simulink model "TCC_MODEL"  (R2025a)
settings: Solver=ode23t  StartTime=0.0  StopTime=1010  FixedStep=0.01  RelTol=1e-3
values from neighbouring files (symbols this model uses):
  HYST = 2    [parametros_componentes.m]
  I_table = [  1.6305773075253425 ... (first row only)    [parametros_componentes.m]
  Icc = -0.000008    (= -8e-06)    [parametros_componentes.m]
  IDD = 25e-6    (= 2.5e-05)    [parametros_componentes.m]
  Ildo = -0.00007    (= -7e-05)    [parametros_componentes.m]
  Iload = 0    [parametros_componentes.m]
  Inicio_da_descarga = 1000    [parametros_componentes.m]
  Inicio_do_curto = 10    [parametros_componentes.m]
  R_curto = 0.5    [parametros_componentes.m]
  R_descarga = (V_BATT_TOTAL+12)/corrente_Max_bat    (= 8.05)    [parametros_componentes.m]
  R_inicial = 0.18    [parametros_componentes.m]
  R_trip = 64.8    [parametros_componentes.m]
  SOC_inicial = 1    [parametros_componentes.m]
  t_table = [  93.22913720326267 ... (first row only)    [parametros_componentes.m]
  tempo_simu_curto = 70    [parametros_componentes.m]
  tempo_simu_descarga = 20    [parametros_componentes.m]
  tempo_simu_temp = 50000    [parametros_componentes.m]
  TSET = 55    [parametros_componentes.m]
  VDD = 3.3    [parametros_componentes.m]
libraries: fl_lib x29, nesl_utility x21, batt_lib x12, ee_lib x2, simulink x1, BatteryEstimators x1
(part 1 of 2)
settings Model: Creator=marce  LastModifiedBy=marce

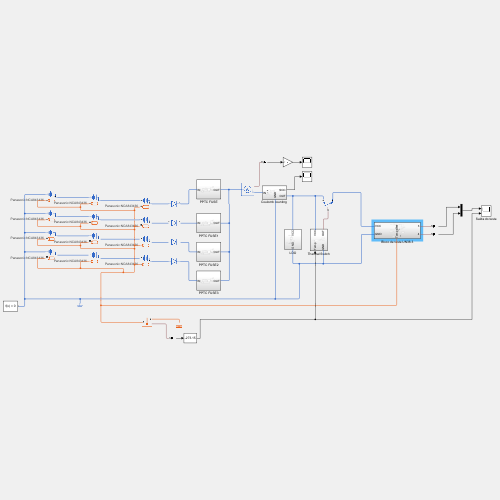
[thumbnail: Simulink's stored preview of the top-level diagram]
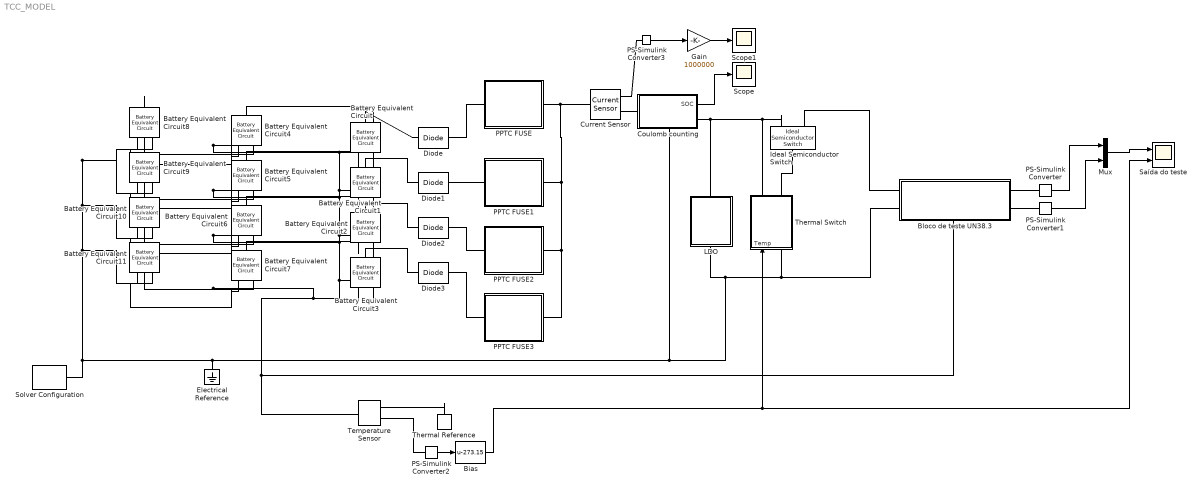
== system TCC_MODEL ==
  Battery Equivalent Circuit : batt_lib/Cells/Battery Equivalent Circuit  PartSpecification="{\"CollectionId\":\"SimscapeBattery\",\"CollectionVersion\":\"1.0.0\",\"DatasetId\":\"Panasonic|NCA843436|simscape.battery.batteryEquivalentCircuit\",\"DisplayName\":\"Panasonic:NCA843436\"}"  BatteryCapacity=1.354 % Datasheet derived hr*A  ThermalModel=simscape.battery.enum.cells.BatteryThermalModel.LumpedThermalMass  ExtrapolationMethod=simscape.enum.extrapolation.linear  SOCBreakpoints=[0 0.01 0.02 0.03 0.04 0.05 0.06 0.07 0.08 0.09 0.1 0.11 0.12 0.13 0.14 0.15 0.16 0.17 0.18 0.19 0.2 0.21 0.22 0.23 0.24 0.25 0.26 0.27 0.28 0.29 0.3 0.31 0.32 0.33 0.34 0.35 0.36 0.37 0.38 0.39 0.4 0.41 0.42 0.43 0.44 0.45 0.46 0.47 0.48 0.49 0.5 0.51 0.52 0.53 0.54 0.55 0.56 0.57 0.58 0.59 0.6 0.61 0.62 0.63 0.64 0.65 0.66 0.67 0.68 0.69 0.7 0.71 0.72 0.73 0.74 0.75 0.76 0.77 0.78 0.79 0.8 0.81 0.82 0.83 0.84 0.85 0.86 0.87 0.88 0.89 0.9 0.91 0.92 0.93 0.94 0.95 0.96 0.97 0.98 0.99 1] % Datasheet derived  TemperatureBreakpoints=[-10 0 10 25 45 60] % Datasheet derived degC  OpenCircuitVoltage=[2.817 2.94537 3.0182 3.08984 3.15197 3.18868 3.22389 3.25188 3.27953 3.3028 3.32214 3.34136 3.36247 3.37682 3.38851 3.4018 3.4147 3.42636 3.43803 3.44822 3.45549 3.46277 3.47005 3.47732 3.4846 3.49328 3.49997 3.50631 3.51243 3.51855 3.52468 3.5308 3.53692 3.54304 3.54917 3.55568 3.56257 3.56948 3.57636 3.58289 3.58942 3.59595 3.60248 3.60901 3.61554 3.62207 3.62861 3.63511 3.64233 3.65 3.65825 3.6665 3.67476 3.68301 3.69126 3.69952 3.70777 3.71583 3.72334 3.73246 3.74258 3.75276 3.76295 3.77313 3.78331 3.7935 3.80368 3.81459 3.82556 3.83654 3.84646 3.85584 3.86522 3.87454 3.8835 3.89255 3.9016 3.91065 3.91971 3.92884 3.93875 3.95021 3.96167 3.97312 3.98443 3.99549 4.00655 4.01783 4.0295 4.04093 4.05161 4.06166 4.07171 4.08185 4.09229 4.10286 4.11335 4.12383 4.13431 4.1515 4.17492] % Datasheet derived V  OpenCircuitVoltageThermal=[2.817 2.817 2.817 2.817 2.817 2.817;2.94537 2.94537 2.94537 2.94537 2.94537 2.94537;3.0182 3.0182 3.0182 3.0182 3.0182 3.0182;3.08984 3.08984 3.08984 3.08984 3.08984 3.08984;3.15197 3.15197 3.15197 3.15197 3.15197 3.15197;3.18868 3.18868 3.18868 3.18868 3.18868 3.18868;3.22389 3.22389 3.22389 3.22389 3.22389 3.22389;3.25188 3.25188 3.25188 3.25188 3.25188 3.25188;3.27953 3.27953 3.27953 3.27953 3.27953 3.27953;3.3028 3.3028 3.3028 3.3028 3.3028 3.3028;3.32214 3.32214 3.32214 3.32214 3.32214 3.32214;3.34136 3.34136 3.34136 3.34136 3.34136 3.34136;3.36247 3.36247 3.36247 3.36247 3.36247 3.36247;3.37682 3.37682 3.37682 3.37682 3.37682 3.37682;3.38851 3.38851 3.38851 3.38851 3.38851 3.38851;3.4018 3.4018 3.4018 3.4018 3.4018 3.4018;3.4147 3.4147 3.4147 3.4147 3.4147 3.4147;3.42636 3.42636 3.42636 3.42636 3.42636 3.42636;3.43803 3.43803 3.43803 3.43803 3.43803 3.43803;3.44822 3.44822 3.44822 3.44822 3.44822 3.44822;3.45549 3.45549 3.45549 3.45549 3.45549 3.45549;3.46277 3.46277 3.46277 3.46277 3.46277 3.46277;3.47005 3.47005 3.47005 3.47005 3.47005 3.47005;3.47732 3.47732 3.47732 3.47732 3.47732 3.47732;3.4846 3.4846 3.4846 3.4846 3.4846 3.4846;3.49328 3.49328 3.49328 3.49328 3.49328 3.49328;3.49997 3.49997 3.49997 3.49997 3.49997 3.49997;3.50631 3.50631 3.50631 3.50631 3.50631 3.50631;3.51243 3.51243 3.51243 3.51243 3.51243 3.51243;3.51855 3.51855 3.51855 3.51855 3.51855 3.51855;3.52468 3.52468 3.52468 3.52468 3.52468 3.52468;3.5308 3.5308 3.5308 3.5308 3.5308 3.5308;3.53692 3.53692 3.53692 3.53692 3.53692 3.53692;3.54304 3.54304 3.54304 3.54304 3.54304 3.54304;3.54917 3.54917 3.54917 3.54917 3.54917 3.54917;3.55568 3.55568 3.55568 3.55568 3.55568 3.55568;3.56257 3.56257 3.56257 3.56257 3.56257 3.56257;3.56948 3.56948 3.56948 3.56948 3.56948 3.56948;3.57636 3.57636 3.57636 3.57636 3.57636 3.57636;3.58289 3.58289 3.58289 3.58289 3.58289 3.58289;3.58942 3.58942 3.58942 3.58942 3.58942 3.58942;3.59595 3.59595 3.59595 3.59595 3.59595 3.59595;3.60248 3.60248 3.60248 3.60248 3.60248 3.60248;3.60901 3.60901 3.60901 3.60901 3.60901 3.60901;3.61554 3.61554 3.61554 3.61554 3.61554 3.61554;3.62207 3.62207 3.62207 3.62207 3.62207 3.62207;3.62861 3.62861 3.62861 3.62861 3.62861 3.62861;3.63511 3.63511 3.63511 3.63511 3.63511 3.63511;3.64233 3.64233 3.64233 3.64233 3.64233 3.64233;3.65 3.65 3.65 3.65 3.65 3.65;3.65825 3.65825 3.65825 3.65825 3.65825 3.65825;3.6665 3.6665 3.6665 3.6665 3.6665 3.6665;3.67476 3.67476 3.67476 3.67476 3.67476 3.67476;3.68301 3.68301 3.68301 3.68301 3.68301 3.68301;3.69126 3.69126 3.69126 3.69126 3.69126 3.69126;3.69952 3.69952 3.69952 3.69952 3.69952 3.69952;3.70777 3.70777 3.70777 3.70777 3.70777 3.70777;3.71583 3.71583 3.71583 3.71583 3.71583 3.71583;3.72334 3.72334 3.72334 3.72334 3.72334 3.72334;3.73246 3.73246 3.73246 3.73246 3.73246 3.73246;3.74258 3.74258 3.74258 3.74258 3.74258 3.74258;3.75276 3.75276 3.75276 3.75276 3.75276 3.75276;3.76295 3.76295 3.76295 3.76295 3.76295 3.76295;3.77313 3.77313 3.77313 3.77313 3.77313 3.77313;3.78331 3.78331 3.78331 3.78331 3.78331 3.78331;3.7935 3.7935 3.7935 3.7935 3.7935 3.7935;3.80368 3.80368 3.80368 3.80368 3.80368 3.80368;3.81459 3.81459 3.81459 3.81459 3.81459 3.81459;3.82556 3.82556 3.82556 3.82556 3.82556 3.82556;3.83654 3.83654 3.83654 3.83654 3.83654 3.83654;3.84646 3.84646 3.84646 3.84646 3.84646 3.84646;3.85584 3.85584 3.85584 3.85584 3.85584 3.85584;3.86522 3.86522 3.86522 3.86522 3.86522 3.86522;3.87454 3.87454 3.87454 3.87454 3.87454 3.87454;3.8835 3.8835 3.8835 3.8835 3.8835 3.8835;3.89255 3.89255 3.89255 3.89255 3.89255 3.89255;3.9016 3.9016 3.9016 3.9016 3.9016 3.9016;3.91065 3.91065 3.91065 3.91065 3.91065 3.91065;3.91971 3.91971 3.91971 3.91971 3.91971 3.91971;3.92884 3.92884 3.92884 3.92884 3.92884 3.92884;3.93875 3.93875 3.93875 3.93875 3.93875 3.93875;3.95021 3.95021 3.95021 3.95021 3.95021 3.95021;3.96167 3.96167 3.96167 3.96167 3.96167 3.96167;3.97312 3.97312 3.97312 3.97312 3.97312 3.97312;3.98443 3.98443 3.98443 3.98443 3.98443 3.98443;3.99549 ...(+748 chars)] % Datasheet derived V  VoltageRange=[2.25 Inf] % Datasheet derived V  HysteresisModel=simscape.battery.enum.cells.HysteresisModel.none  MaximumHysteresisVoltage=[0, 0, 0, 0, 0, 0, 0] % Parameter not set V  InstantaneousHysteresisVoltage=[0, 0, 0, 0, 0, 0, 0] % Parameter not set V  HysteresisRate=0.1 % Parameter not set  MaximumHysteresisVoltageThermal=[0, 0, 0; 0, 0, 0; 0, 0, 0; 0, 0, 0; 0, 0, 0; 0, 0, 0; 0, 0, 0] % Parameter not set V  InstantaneousHysteresisVoltageThermal=[0, 0, 0; 0, 0, 0; 0, 0, 0; 0, 0, 0; 0, 0, 0; 0, 0, 0; 0, 0, 0] % Parameter not set V  HysteresisRateThermal=0.1 % Parameter not set  ResistanceSOCBreakpoints=[0 0.01 0.02 0.03 0.04 0.05 0.06 0.07 0.08 0.09 0.1 0.11 0.12 0.13 0.14 0.15 0.16 0.17 0.18 0.19 0.2 0.21 0.22 0.23 0.24 0.25 0.26 0.27 0.28 0.29 0.3 0.31 0.32 0.33 0.34 0.35 0.36 0.37 0.38 0.39 0.4 0.41 0.42 0.43 0.44 0.45 0.46 0.47 0.48 0.49 0.5 0.51 0.52 0.53 0.54 0.55 0.56 0.57 0.58 0.59 0.6 0.61 0.62 0.63 0.64 0.65 0.66 0.67 0.68 0.69 0.7 0.71 0.72 0.73 0.74 0.75 0.76 0.77 0.78 0.79 0.8 0.81 0.82 0.83 0.84 0.85 0.86 0.87 0.88 0.89 0.9 0.91 0.92 0.93 0.94 0.95 0.96 0.97 0.98 0.99 1] % Datasheet derived  ResistanceTemperatureBreakpoints=[-10 0 10 25 45 60] % Datasheet derived degC  ResistanceCurrentBreakpoints=[-1, 0, 1] % Parameter not set A  CurrentDependence=simscape.battery.enum.cells.CurrentDependence.Disabled  R0=[0.31638 0.3243 0.30647 0.2881 0.26534 0.23483 0.21466 0.1963 0.19065 0.18321 0.17517 0.17035 0.1686 0.16602 0.16263 0.16182 0.16098 0.16003 0.15908 0.15746 0.15485 0.15224 0.14963 0.14702 0.14441 0.14408 0.14309 0.14204 0.14098 0.13992 0.13886 0.13779 0.13673 0.13567 0.13461 0.13373 0.13328 0.13287 0.13246 0.13202 0.13158 0.13114 0.1307 0.13026 0.12982 0.12938 0.12894 0.12846 0.12829 0.12823 0.12821 0.1282 0.12818 0.12817 0.12815 0.12814 0.12812 0.12779 0.12659 0.12613 0.1261 0.12607 0.12605 0.12602 0.126 0.12598 0.12595 0.12709 0.12835 0.1296 0.13037 0.13088 0.1314 0.13182 0.13158 0.13136 0.13113 0.1309 0.13069 0.13059 0.13086 0.13184 0.13283 0.13381 0.13455 0.1349 0.13525 0.13561 0.13601 0.1363 0.13601 0.1347 0.13339 0.13211 0.13099 0.12903 0.12626 0.1235 0.12073 0.11181 0.10295] % Datasheet derived Ohm  R0I=[.0117, .0085, .009; .011, .0085, .009; .0114, .0087, .0092; .0107, .0082, .0088; .0107, .0083, .0091; .0113, .0085, .0089; .0116, .0085, .0089] % Parameter not set Ohm  R0Thermal=[1.5461 1.75516 2.11759 0.31638 0.46651 0.23498;1.5461 1.99954 2.27305 0.3243 0.34615 0.09965;1.5461 1.92281 2.1374 0.30647 0.20343 0.05211;1.5461 1.84609 2.00176 0.2881 0.15069 0.02648;1.5461 1.76937 1.86611 0.26534 0.12351 0.03545;1.5461 1.69264 1.73046 0.23483 0.10579 0.0319;1.5461 1.61592 1.59482 0.21466 0.09923 0.03983;1.5461 1.5392 1.45917 0.1963 0.0958 0.05105;1.5461 1.46247 1.32352 0.19065 0.10282 0.06344;1.5461 1.38575 1.18787 0.18321 0.10641 0.07241;1.5461 1.30902 1.05223 0.17517 0.10811 0.07828;1.5461 1.2323 0.91658 0.17035 0.11082 0.08499;1.5461 1.15558 0.78093 0.1686 0.11501 0.09321;1.50339 1.07885 0.64529 0.16602 0.11389 0.09611;1.46067 1.00213 0.52896 0.16263 0.11281 0.09693;1.41796 0.92541 0.45732 0.16182 0.1148 0.09886;1.37525 0.84868 0.40356 0.16098 0.11649 0.10041;1.33254 0.77196 0.35633 0.16003 0.1172 0.10099;1.28982 0.69523 0.32513 0.15908 0.11792 0.10158;1.24711 0.61749 0.29756 0.15746 0.11748 0.101;1.2044 0.5576 0.27681 0.15485 0.11475 0.09814;1.16169 0.50708 0.25953 0.15224 0.11202 0.09528;1.11897 0.46758 0.24304 0.14963 0.11054 0.09242;1.07626 0.43256 0.23145 0.14702 0.10939 0.09016;1.03355 0.40213 0.21986 0.14441 0.10825 0.08946;0.99084 0.37836 0.21479 0.14408 0.10821 0.08986;0.94812 0.35585 0.21092 0.14309 0.1066 0.08869;0.90541 0.33652 0.20677 0.14204 0.10481 0.08725;0.8627 0.32218 0.20275 0.14098 0.10391 0.08564;0.81999 0.30785 0.19912 0.13992 0.10301 0.08404;0.77727 0.29756 0.19549 0.13886 0.1021 0.08274;0.73457 0.28818 0.19186 0.13779 0.10125 0.08295;0.69186 0.2788 0.1889 0.13673 0.10088 0.08317;0.65043 0.27154 0.18649 0.13567 0.10051 0.08339;0.60913 0.26481 0.18408 0.13461 0.10013 0.0836;0.57538 0.25838 0.18198 0.13373 0.10007 0.08413;0.5481 0.25225 0.18022 0.13328 0.10029 0.08494;0.52084 0.24869 0.17996 0.13287 0.10054 0.08577;0.49467 0.24569 0.17968 0.13246 0.10076 0.08658;0.47265 0.24242 0.17912 0.13202 0.10071 0.08711;0.45063 0.23914 0.17856 0.13158 0.10065 0.08708;0.43278 0.23587 0.17801 0.13114 0.10056 0.08706;0.42113 0.23372 0.17745 0.1307 0.09993 0.08703;0.40948 0.23194 0.17689 0.13026 0.09931 0.087;0.39802 0.23016 0.17625 0.12982 0.09869 0.08698;0.3895 0.22838 0.17554 0.12938 0.09807 0.08695;0.38098 0.2266 0.17484 0.12894 0.09745 0.08692;0.37243 0.2248 0.17411 0.12846 0.09681 0.08688;0.36446 0.22399 0.17395 0.12829 0.09673 0.08739;0.35683 0.2238 0.17413 0.12823 0.097 0.08826;0.35467 0.22407 0.17478 0.12821 0.09771 0.08958;0.35251 0.22433 0.17543 0.1282 0.098 0.09079;0.35035 0.2246 0.17607 0.12818 0.09829 0.09028;0.34819 0.22487 0.17654 0.12817 0.09857 0.08977;0.34604 0.22513 0.17577 0.12815 0.09886 0.08925;0.34388 0.2254 0.175 0.12814 0.09915 0.08874;0.34172 0.22541 0.17423 0.12812 0.09944 0.08823;0.3394 0.22519 0.17331 0.12779 0.09957 0.08756;0.33667 0.22454 0.17196 0.12659 0.09928 0.08647;0.33518 0.22514 0.17187 0.12613 0.10014 0.08664;0.33524 0.22653 0.17256 0.1261 0.10082 0.08759;0.33556 0.22797 0.1733 0.12607 0.10155 0.0885;0.33589 0.22941 0.17405 0.12605 0.10227 0.08918;0.33622 0.23086 0.17484 0.12602 0.103 0.08985;0.33655 0.2323 0.1758 0.126 0.10373 0.09053;0.33688 0.23374 0.17676 0.12598 0.10446 0.0912;0.33721 0.23499 0.17772 0.12595 0.10519 0.09188;0.3381 0.23639 0.17924 0.12709 0.10648 0.09312;0.33905 0.23784 0.18082 0.12835 0.10783 0.09441;0.34 0.23929 0.18241 0.1296 0.10918 0.09571;0.34031 0.23991 0.18316 0.13037 0.1097 0.09618;0.34036 0.24011 0.18349 0.13088 0.1098 0.09608;0.3404 0.24031 0.18382 0.1314 0.10989 0.09597;0.3404 0.24047 0.1841 0.13182 0.10986 0.09581;0.34011 0.24033 0.1841 0.13158 0.10953 0.09535;0.33989 0.24027 0.18422 0.13136 0.10929 0.09498;0.34006 0.24021 0.18463 0.13113 0.10904 0.09461;0.34112 0.24015 0.18505 0.1309 0.1088 0.09423;0.34219 0.24057 0.18547 0.13069 0.10855 0.09385;0.34331 0.24158 0.18594 0.13059 0.10837 0.09322;0.34505 0.2432 0.18703 0.13086 0.10748 0.0932;0.348 0.24604 0.18933 0.13184 0.10774 0.09438;0.35095 0.24887 0.19163 0.13283 0.108 0.09557;0.35389 0.25171 0.19393 0.13381 0.10826 0.09676;0.35814 0.25442 0.19611 0.13455 0.1084 0.09783 ...(+755 chars)] % Datasheet derived Ohm  R0ThermalI=repmat([.0117, .0085, .009; .011, .0085, .009; .0114, .0087, .0092; .0107, .0082, .0088; .0107, .0083, .0091; .0113, .0085, .0089; .0116, .0085, .0089], 1, 1, 3) % Parameter not set Ohm  DischargeR0=[.0085, .0085, .0087, .0082, .0083, .0085, .0085] % Parameter not set Ohm  ChargeR0=[.0085, .0085, .0087, .0082, .0083, .0085, .0085] % Parameter not set Ohm  ChargeR0Thermal=[.0117, .0085, .009; .011, .0085, .009; .0114, .0087, .0092; .0107, .0082, .0088; .0107, .0083, .0091; .0113, .0085, .0089; .0116, .0085, .0089] % Parameter not set Ohm  DischargeR0Thermal=[.0117, .0085, .009; .011, .0085, .009; .0114, .0087, .0092; .0107, .0082, .0088; .0107, .0083, .0091; .0113, .0085, .0089; .0116, .0085, .0089] % Parameter not set Ohm  RCPairs=simscape.battery.enum.cells.RCPairs.noDynamics  R1=[.0029, .0024, .0026, .0016, .0023, .0018, .0017] % Parameter not set Ohm  Tau1=[36, 45, 105, 29, 77, 33, 39] % Parameter not set s  R2=[.0029, .0024, .0026, .0016, .0023, .0018, .0017] % Parameter not set Ohm  Tau2=[36, 45, 105, 29, 77, 33, 39] % Parameter not set s  R3=[.0029, .0024, .0026, .0016, .0023, .0018, .0017] % Parameter not set Ohm  Tau3=[36, 45, 105, 29, 77, 33, 39] % Parameter not set s  R1I=[.0109, .0029, .0013; .0069, .0024, .0012; .0047, .0026, .0013; .0034, .0016, .001; .0033, .0023, .0014; .0033, .0018, .0011; .0028, .0017, .0011] % Parameter not set Ohm  Tau1I=[20, 36, 39; 31, 45, 39; 109, 105, 61; 36, 29, 26; 59, 77, 67; 40, 33, 29; 25, 39, 33] % Parameter not set s  R2I=[.0109, .0029, .0013; .0069, .0024, .0012; .0047, .0026, .0013; .0034, .0016, .001; .0033, .0023, .0014; .0033, .0018, .0011; .0028, .0017, .0011] % Parameter not set Ohm  Tau2I=[20, 36, 39; 31, 45, 39; 109, 105, 61; 36, 29, 26; 59, 77, 67; 40, 33, 29; 25, 39, 33] % Parameter not set s  R3I=[.0109, .0029, .0013; .0069, .0024, .0012; .0047, .0026, .0013; .0034, .0016, .001; .0033, .0023, .0014; .0033, .0018, .0011; .0028, .0017, .0011] % Parameter not set Ohm  Tau3I=[20, 36, 39; 31, 45, 39; 109, 105, 61; 36, 29, 26; 59, 77, 67; 40, 33, 29; 25, 39, 33] % Parameter not set s  DischargeR1=[.0029, .0024, .0026, .0016, .0023, .0018, .0017] % Parameter not set Ohm  DischargeTau1=[36, 45, 105, 29, 77, 33, 39] % Parameter not set s  ChargeR1=[.0029, .0024, .0026, .0016, .0023, .0018, .0017] % Parameter not set Ohm  ChargeTau1=[36, 45, 105, 29, 77, 33, 39] % Parameter not set s  DischargeR2=[.0029, .0024, .0026, .0016, .0023, .0018, .0017] % Parameter not set Ohm  DischargeTau2=[36, 45, 105, 29, 77, 33, 39] % Parameter not set s  ChargeR2=[.0029, .0024, .0026, .0016, .0023, .0018, .0017] % Parameter not set Ohm  ChargeTau2=[36, 45, 105, 29, 77, 33, 39] % Parameter not set s  DischargeR3=[.0029, .0024, .0026, .0016, .0023, .0018, .0017] % Parameter not set Ohm  DischargeTau3=[36, 45, 105, 29, 77, 33, 39] % Parameter not set s  ChargeR3=[.0029, .0024, .0026, .0016, .0023, .0018, .0017] % Parameter not set Ohm  ChargeTau3=[36, 45, 105, 29, 77, 33, 39] % Parameter not set s  R1Thermal=[.0109, .0029, .0013; .0069, .0024, .0012; .0047, .0026, .0013; .0034, .0016, .001; .0033, .0023, .0014; .0033, .0018, .0011; .0028, .0017, .0011] % Parameter not set Ohm  Tau1Thermal=[20, 36, 39; 31, 45, 39; 109, 105, 61; 36, 29, 26; 59, 77, 67; 40, 33, 29; 25, 39, 33] % Parameter not set s  R2Thermal=[.0109, .0029, .0013; .0069, .0024, .0012; .0047, .0026, .0013; .0034, .0016, .001; .0033, .0023, .0014; .0033, .0018, .0011; .0028, .0017, .0011] % Parameter not set Ohm  Tau2Thermal=[20, 36, 39; 31, 45, 39; 109, 105, 61; 36, 29, 26; 59, 77, 67; 40, 33, 29; 25, 39, 33] % Parameter not set s  R3Thermal=[.0109, .0029, .0013; .0069, .0024, .0012; .0047, .0026, .0013; .0034, .0016, .001; .0033, .0023, .0014; .0033, .0018, .0011; .0028, .0017, .0011] % Parameter not set Ohm  Tau3Thermal=[20, 36, 39; 31, 45, 39; 109, 105, 61; 36, 29, 26; 59, 77, 67; 40, 33, 29; 25, 39, 33] % Parameter not set s  R1ThermalI=repmat([.0109, .0029, .0013; .0069, .0024, .0012; .0047, .0026, .0013; .0034, .0016, .001; .0033, .0023, .0014; .0033, .0018, .0011; .0028, .0017, .0011], 1, 1, 3) % Parameter not set Ohm  Tau1ThermalI=repmat([20, 36, 39; 31, 45, 39; 109, 105, 61; 36, 29, 26; 59, 77, 67; 40, 33, 29; 25, 39, 33], 1, 1, 3) % Parameter not set s  R2ThermalI=repmat([.0109, .0029, .0013; .0069, .0024, .0012; .0047, .0026, .0013; .0034, .0016, .001; .0033, .0023, .0014; .0033, .0018, .0011; .0028, .0017, .0011], 1, 1, 3) % Parameter not set Ohm  Tau2ThermalI=repmat([20, 36, 39; 31, 45, 39; 109, 105, 61; 36, 29, 26; 59, 77, 67; 40, 33, 29; 25, 39, 33], 1, 1, 3) % Parameter not set s  R3ThermalI=repmat([.0109, .0029, .0013; .0069, .0024, .0012; .0047, .0026, .0013; .0034, .0016, .001; .0033, .0023, .0014; .0033, .0018, .0011; .0028, .0017, .0011], 1, 1, 3) % Parameter not set Ohm  Tau3ThermalI=repmat([20, 36, 39; 31, 45, 39; 109, 105, 61; 36, 29, 26; 59, 77, 67; 40, 33, 29; 25, 39, 33], 1, 1, 3) % Parameter not set s  DischargeR1Thermal=[.0109, .0029, .0013; .0069, .0024, .0012; .0047, .0026, .0013; .0034, .0016, .001; .0033, .0023, .0014; .0033, .0018, .0011; .0028, .0017, .0011] % Parameter not set Ohm  DischargeTau1Thermal=[20, 36, 39; 31, 45, 39; 109, 105, 61; 36, 29, 26; 59, 77, 67; 40, 33, 29; 25, 39, 33] % Parameter not set s  ChargeR1Thermal=[.0109, .0029, .0013; .0069, .0024, .0012; .0047, .0026, .0013; .0034, .0016, .001; .0033, .0023, .0014; .0033, .0018, .0011; .0028, .0017, .0011] % Parameter not set Ohm  ChargeTau1Thermal=[20, 36, 39; 31, 45, 39; 109, 105, 61; 36, 29, 26; 59, 77, 67; 40, 33, 29; 25, 39, 33] % Parameter not set s  DischargeR2Thermal=[.0109, .0029, .0013; .0069, .0024, .0012; .0047, .0026, .0013; .0034, .0016, .001; .0033, .0023, .0014; .0033, .0018, .0011; .0028, .0017, .0011] % Parameter not set Ohm  DischargeTau2Thermal=[20, 36, 39; 31, 45, 39; 109, 105, 61; 36, 29, 26; 59, 77, 67; 40, 33, 29; 25, 39, 33] % Parameter not set s  ChargeR2Thermal=[.0109, .0029, .0013; .0069, .0024, .0012; .0047, .0026, .0013; .0034, .0016, .001; .0033, .0023, .0014; .0033, .0018, .0011; .0028, .0017, .0011] % Parameter not set Ohm  ChargeTau2Thermal=[20, 36, 39; 31, 45, 39; 109, 105, 61; 36, 29, 26; 59, 77, 67; 40, 33, 29; 25, 39, 33] % Parameter not set s  DischargeR3Thermal=[.0109, .0029, .0013; .0069, .0024, .0012; .0047, .0026, .0013; .0034, .0016, .001; .0033, .0023, .0014; .0033, .0018, .0011; .0028, .0017, .0011] % Parameter not set Ohm  DischargeTau3Thermal=[20, 36, 39; 31, 45, 39; 109, 105, 61; 36, 29, 26; 59, 77, 67; 40, 33, 29; 25, 39, 33] % Parameter not set s  ChargeR3Thermal=[.0109, .0029, .0013; .0069, .0024, .0012; .0047, .0026, .0013; .0034, .0016, .001; .0033, .0023, .0014; .0033, .0018, .0011; .0028, .0017, .0011] % Parameter not set Ohm  ChargeTau3Thermal=[20, 36, 39; 31, 45, 39; 109, 105, 61; 36, 29, 26; 59, 77, 67; 40, 33, 29; 25, 39, 33] % Parameter not set s  SelfDischargeResistor=simscape.battery.enum.cells.BatteryEnable.Disabled  SelfDischargeR=7e3 % Parameter not set Ohm  SelfDischargeRThermal=[8000, 7000, 6000] % Parameter not set Ohm  CyclingAgingMethod=simscape.battery.enum.cells.CyclingAgingMethod.tableN  CycleCalculationMethod=simscape.battery.enum.cells.CycleCalculationMethod.EquivalentCycles  NumDisCycles=100 % Parameter not set  OCVChange=0 % Parameter not set  R0Change=0 % Parameter not set  CapacityChange=0 % Parameter not set  SelfDischargeRChange=0 % Parameter not set  R1Change=0 % Parameter not set  R2Change=0 % Parameter not set  R3Change=0 % Parameter not set  NumDisCyclesBreakpoints=[0 7 13 19 25 31 37 43 49 55 61 67 73 79 85 91 97 103 109 115 121 127 133 139 145 151 157 163 169 175 181 187 193 199 205 211 217 223 229 235 241 247 253 259 265 271 277 283 289 295 301 307 313 319 325 331 337 343 349 355 361 367 373 379 385 391 397 403 409 415 421 427 433 439 445 451 457 463 469 475 481 487 493 499] % Datasheet derived  AgingTemperatureBreakpoints=[298.15, 323.15] % Parameter not set K  AgingCurrentBreakpoints=[-.1, -.5, -5] % Parameter not set A  OCVChangeVec=[0 -0.2056 -0.4112 -0.602 -0.7529 -0.9041 -1.0234 -1.116 -1.2087 -1.3013 -1.3939 -1.4865 -1.5404 -1.5936 -1.6468 -1.7 -1.7534 -1.807 -1.8607 -1.9143 -1.972 -2.0316 -2.0912 -2.1507 -2.2103 -2.2687 -2.3264 -2.3842 -2.442 -2.4996 -2.5474 -2.5914 -2.6354 -2.6795 -2.7235 -2.7676 -2.8116 -2.8556 -2.8997 -2.9437 -2.9899 -3.057 -3.1273 -3.1975 -3.2718 -3.347 -3.4222 -3.4977 -3.5744 -3.6428 -3.6945 -3.7461 -3.7966 -3.8466 -3.8965 -3.9465 -3.9964 -4.0461 -4.0951 -4.1498 -4.2072 -4.2646 -4.322 -4.3794 -4.4368 -4.4942 -4.5515 -4.61 -4.6685 -4.7269 -4.7854 -4.844 -4.9032 -4.9624 -5.0216 -5.0808 -5.1413 -5.2041 -5.2668 -5.3295 -5.3922 -5.455 -5.5177 -5.5804] % Datasheet derived  OCVChangeThermal=[0, 0; 0, 0; 0, 0; 0, 0] % Parameter not set  R0ChangeVec=[0 0 0 0 0 0 0 0 0 0 0 0 0 0 0 0 0 0 0 0 0 0 0 0 0 0 0 0 0 0 0 0 0 0 0 0 0 0 0 0 0 0 0 0 0 0 0 0 0 0 0 0 0 0 0 0 0 0 0 0 0 0 0 0 0 0 0 0 0 0 0 0 0 0 0 0 0 0 0 0 0 0 0 0] % Parameter assumed  R0ChangeThermal=[0, 0; 0, 0; 0, 0; 0, 0] % Parameter not set  R0ChangeThermalI=repmat(0, 4, 2, 3) % Parameter not set  R0CyclingChangeInitialTarget=0 % Parameter not set  CapacityChangeVec=[0 -0.367 -0.733 -1.1 -1.466 -1.834 -2.202 -2.571 -2.94 -3.309 -3.678 -4.047 -4.261 -4.473 -4.685 -4.897 -5.109 -5.32 -5.532 -5.744 -5.972 -6.21 -6.448 -6.686 -6.924 -7.162 -7.4 -7.638 -7.876 -8.114 -8.313 -8.496 -8.679 -8.862 -9.045 -9.228 -9.411 -9.593 -9.776 -9.959 -10.142 -10.405 -10.679 -10.954 -11.228 -11.503 -11.777 -12.052 -12.326 -12.571 -12.756 -12.941 -13.126 -13.311 -13.496 -13.681 -13.866 -14.051 -14.235 -14.442 -14.659 -14.875 -15.092 -15.308 -15.525 -15.741 -15.958 -16.175 -16.391 -16.607 -16.822 -17.038 -17.254 -17.47 -17.685 -17.901 -18.122 -18.35 -18.579 -18.807 -19.036 -19.265 -19.493 -19.722] % Datasheet derived  CapacityChangeThermal=[0, 0; 0, 0; 0, 0; 0, 0] % Parameter not set  CapacityChangeThermalI=repmat(0, 4, 2, 3) % Parameter not set  CapacityCyclingChangeInitialTarget=0 % Parameter not set  SelfDischargeRChangeVec=[0, 0, 0, 0] % Parameter not set  SelfDischargeRChangeThermal=[0, 0; 0, 0; 0, 0; 0, 0] % Parameter not set  SelfDischargeRChangeThermalI=repmat(0, 4, 2, 3) % Parameter not set  SelfDischargeRCyclingChangeInitialTarget=0 % Parameter not set  R1ChangeVec=[0, 0, 0, 0] % Parameter not set  R1ChangeThermal=[0, 0; 0, 0; 0, 0; 0, 0] % Parameter not set  R1ChangeThermalI=repmat(0, 4, 2, 3) % Parameter not set  R1CyclingChangeInitialTarget=0 % Parameter not set  R2ChangeVec=[0, 0, 0, 0] % Parameter not set  R2ChangeThermal=[0, 0; 0, 0; 0, 0; 0, 0] % Parameter not set  R2ChangeThermalI=repmat(0, 4, 2, 3) % Parameter not set  R2CyclingChangeInitialTarget=0 % Parameter not set  R3ChangeVec=[0, 0, 0, 0] % Parameter not set  R3ChangeThermal=[0, 0; 0, 0; 0, 0; 0, 0] % Parameter not set  R3ChangeThermalI=repmat(0, 4, 2, 3) % Parameter not set  R3CyclingChangeInitialTarget=0 % Parameter not set  CalendarAgeResistance=simscape.battery.enum.cells.BatteryEnable.Disabled  CalendarAgeCapacity=simscape.battery.enum.cells.BatteryEnable.Disabled  CalendarAgingMethod=simscape.battery.enum.cells.CalendarAgingMethod.equation  StorageVariable=simscape.battery.enum.cells.StorageVariable.OCV  OCVDuringStorage=0.9 % Parameter not set  SOCDuringStorage=0.6 % Parameter not set  StorageTimeIntervals=[0] % Parameter not set d  StorageTemperatures=[273] % Parameter not set K  ResistanceScalingOCV=2.2134e6 % Parameter not set  ResistanceScalingOCVOffset=1.632e6 % Parameter not set  ResistanceExponentialIncrease=0.515833569 % Parameter not set V  ResistanceTimeExponent=0.75 % Parameter not set  ResistanceAgeTemperatureBreakpoints=[273.15, 298.15, 323.15] % Parameter not set K  ResistanceAgeTimeBreakpoints=[0, 90, 180, 270] % Parameter not set d  PercentResistanceChange=[0, 0, 0] % Parameter not set  ResistanceTimeBreakpoints=100 % Parameter not set d  PercentResistanceChangeThermal=[0, 0, 0; 0, 0, 0; 0, 0, 0; 0, 0, 0] % Parameter not set  CapacityScalingOCV=1.5097e07 % Parameter not set  CapacityScalingOCVOffset=8.3625e06 % Parameter not set  CapacityExponentialIncrease=0.6011 % Parameter not set V  CapacityTimeExponent=0.75 % Parameter not set  CapacityAgeTemperatureBreakpoints=[273.15, 298.15, 323.15] % Parameter not set K  CapacityAgeTimeBreakpoints=[0, 90, 180, 270] % Parameter not set d  PercentCapacityChange=[0, 0, 0] % Parameter not set  CapacityTimeBreakpoints=100 % Parameter not set d  PercentCapacityChangeThermal=[0, 0, 0; 0, 0, 0; 0, 0, 0; 0, 0, 0] % Parameter not set  SimulationTemperature=298.15 % Parameter not set K  BatteryThermalMass=20.7 % Parameter assumed J/K  NumThermalModels=6 % Parameter not set  ThermalConductivityZ=18 % Parameter not set W/(K*m)  CrossSectionalAreaXY=0.000286 m^2  Height=0.036 m  ReversibleHeatModel=simscape.battery.enum.cells.ReversibleHeatModel.Disabled  EntropicCoefficient=[0, 0, 0, 0, 0, 0, 0] % Parameter not set mV/K  CurrentDirectionality=simscape.battery.enum.cells.BatteryEnable.Disabled  stateOfCharge_specify=off  stateOfCharge_priority=High  stateOfCharge=1  stateOfCharge_nominal_specify=off  stateOfCharge_nominal_value=1  stateOfCharge_nominal_unit=1  batteryVoltage_specify=off  batteryVoltage_priority=Low  batteryVoltage=3 V  batteryVoltage_nominal_specify=off  batteryVoltage_nominal_value=1  batteryVoltage_nominal_unit=V  batteryCurrent_specify=off  batteryCurrent_priority=None  batteryCurrent=0 A  batteryCurrent_nominal_specify=off  batteryCurrent_nominal_value=1  batteryCurrent_nominal_unit=A  numCycles_specify=off  numCycles_priority=High  numCycles=0  numCycles_nominal_specify=off  numCycles_nominal_value=1  numCycles_nominal_unit=1  batteryTemperature_specify=off  batteryTemperature_priority=High  batteryTemperature=298.15 K  batteryTemperature_nominal_specify=off  batteryTemperature_nominal_value=1  batteryTemperature_nominal_unit=K  hysteresisState_specify=off  hysteresisState_priority=High  hysteresisState=0  hysteresisState_nominal_specify=off  hysteresisState_nominal_value=1  hysteresisState_nominal_unit=1  isExothermFaulted_specify=off  isExothermFaulted_priority=None  isExothermFaulted=0  isExothermFaulted_nominal_specify=off  isExothermFaulted_nominal_value=1  isExothermFaulted_nominal_unit=1  reactionHeatRate_specify=off  reactionHeatRate_priority=None  reactionHeatRate=0 W  reactionHeatRate_nominal_specify=off  reactionHeatRate_nominal_value=1  reactionHeatRate_nominal_unit=W  reactionExtent_specify=off  reactionExtent_priority=None  reactionExtent=0  reactionExtent_nominal_specify=off  reactionExtent_nominal_value=1  reactionExtent_nominal_unit=1
      settings: AttributesFormatString=Panasonic:NCA843436  InternalSimscapePortConfiguration="{\"Bottom\":[{\"id\":\"n\",\"label\":\"-\",\"type\":\"foundation.electrical.electrical\"},{\"id\":\"H\",\"label\":\"H\",\"type\":\"foundation.thermal.thermal\"}],\"Left\":[],\"Right\":[],\"Top\":[{\"id\":\"p\",\"label\":\"+\",\"type\":\"foundation.electrical.electrical\"}]}"
  Battery Equivalent Circuit{1..3,5..7,9..11} (9 alike) : batt_lib/Cells/Battery Equivalent Circuit  PartSpecification="{\"CollectionId\":\"SimscapeBattery\",\"CollectionVersion\":\"1.0.0\",\"DatasetId\":\"Panasonic|NCA843436|simscape.battery.batteryEquivalentCircuit\",\"DisplayName\":\"Panasonic:NCA843436\"}"  BatteryCapacity=1.354 % Datasheet derived hr*A  ThermalModel=simscape.battery.enum.cells.BatteryThermalModel.LumpedThermalMass  ExtrapolationMethod=simscape.enum.extrapolation.linear  SOCBreakpoints=[0 0.01 0.02 0.03 0.04 0.05 0.06 0.07 0.08 0.09 0.1 0.11 0.12 0.13 0.14 0.15 0.16 0.17 0.18 0.19 0.2 0.21 0.22 0.23 0.24 0.25 0.26 0.27 0.28 0.29 0.3 0.31 0.32 0.33 0.34 0.35 0.36 0.37 0.38 0.39 0.4 0.41 0.42 0.43 0.44 0.45 0.46 0.47 0.48 0.49 0.5 0.51 0.52 0.53 0.54 0.55 0.56 0.57 0.58 0.59 0.6 0.61 0.62 0.63 0.64 0.65 0.66 0.67 0.68 0.69 0.7 0.71 0.72 0.73 0.74 0.75 0.76 0.77 0.78 0.79 0.8 0.81 0.82 0.83 0.84 0.85 0.86 0.87 0.88 0.89 0.9 0.91 0.92 0.93 0.94 0.95 0.96 0.97 0.98 0.99 1] % Datasheet derived  TemperatureBreakpoints=[-10 0 10 25 45 60] % Datasheet derived degC  OpenCircuitVoltage=[2.817 2.94537 3.0182 3.08984 3.15197 3.18868 3.22389 3.25188 3.27953 3.3028 3.32214 3.34136 3.36247 3.37682 3.38851 3.4018 3.4147 3.42636 3.43803 3.44822 3.45549 3.46277 3.47005 3.47732 3.4846 3.49328 3.49997 3.50631 3.51243 3.51855 3.52468 3.5308 3.53692 3.54304 3.54917 3.55568 3.56257 3.56948 3.57636 3.58289 3.58942 3.59595 3.60248 3.60901 3.61554 3.62207 3.62861 3.63511 3.64233 3.65 3.65825 3.6665 3.67476 3.68301 3.69126 3.69952 3.70777 3.71583 3.72334 3.73246 3.74258 3.75276 3.76295 3.77313 3.78331 3.7935 3.80368 3.81459 3.82556 3.83654 3.84646 3.85584 3.86522 3.87454 3.8835 3.89255 3.9016 3.91065 3.91971 3.92884 3.93875 3.95021 3.96167 3.97312 3.98443 3.99549 4.00655 4.01783 4.0295 4.04093 4.05161 4.06166 4.07171 4.08185 4.09229 4.10286 4.11335 4.12383 4.13431 4.1515 4.17492] % Datasheet derived V  OpenCircuitVoltageThermal=[2.817 2.817 2.817 2.817 2.817 2.817;2.94537 2.94537 2.94537 2.94537 2.94537 2.94537;3.0182 3.0182 3.0182 3.0182 3.0182 3.0182;3.08984 3.08984 3.08984 3.08984 3.08984 3.08984;3.15197 3.15197 3.15197 3.15197 3.15197 3.15197;3.18868 3.18868 3.18868 3.18868 3.18868 3.18868;3.22389 3.22389 3.22389 3.22389 3.22389 3.22389;3.25188 3.25188 3.25188 3.25188 3.25188 3.25188;3.27953 3.27953 3.27953 3.27953 3.27953 3.27953;3.3028 3.3028 3.3028 3.3028 3.3028 3.3028;3.32214 3.32214 3.32214 3.32214 3.32214 3.32214;3.34136 3.34136 3.34136 3.34136 3.34136 3.34136;3.36247 3.36247 3.36247 3.36247 3.36247 3.36247;3.37682 3.37682 3.37682 3.37682 3.37682 3.37682;3.38851 3.38851 3.38851 3.38851 3.38851 3.38851;3.4018 3.4018 3.4018 3.4018 3.4018 3.4018;3.4147 3.4147 3.4147 3.4147 3.4147 3.4147;3.42636 3.42636 3.42636 3.42636 3.42636 3.42636;3.43803 3.43803 3.43803 3.43803 3.43803 3.43803;3.44822 3.44822 3.44822 3.44822 3.44822 3.44822;3.45549 3.45549 3.45549 3.45549 3.45549 3.45549;3.46277 3.46277 3.46277 3.46277 3.46277 3.46277;3.47005 3.47005 3.47005 3.47005 3.47005 3.47005;3.47732 3.47732 3.47732 3.47732 3.47732 3.47732;3.4846 3.4846 3.4846 3.4846 3.4846 3.4846;3.49328 3.49328 3.49328 3.49328 3.49328 3.49328;3.49997 3.49997 3.49997 3.49997 3.49997 3.49997;3.50631 3.50631 3.50631 3.50631 3.50631 3.50631;3.51243 3.51243 3.51243 3.51243 3.51243 3.51243;3.51855 3.51855 3.51855 3.51855 3.51855 3.51855;3.52468 3.52468 3.52468 3.52468 3.52468 3.52468;3.5308 3.5308 3.5308 3.5308 3.5308 3.5308;3.53692 3.53692 3.53692 3.53692 3.53692 3.53692;3.54304 3.54304 3.54304 3.54304 3.54304 3.54304;3.54917 3.54917 3.54917 3.54917 3.54917 3.54917;3.55568 3.55568 3.55568 3.55568 3.55568 3.55568;3.56257 3.56257 3.56257 3.56257 3.56257 3.56257;3.56948 3.56948 3.56948 3.56948 3.56948 3.56948;3.57636 3.57636 3.57636 3.57636 3.57636 3.57636;3.58289 3.58289 3.58289 3.58289 3.58289 3.58289;3.58942 3.58942 3.58942 3.58942 3.58942 3.58942;3.59595 3.59595 3.59595 3.59595 3.59595 3.59595;3.60248 3.60248 3.60248 3.60248 3.60248 3.60248;3.60901 3.60901 3.60901 3.60901 3.60901 3.60901;3.61554 3.61554 3.61554 3.61554 3.61554 3.61554;3.62207 3.62207 3.62207 3.62207 3.62207 3.62207;3.62861 3.62861 3.62861 3.62861 3.62861 3.62861;3.63511 3.63511 3.63511 3.63511 3.63511 3.63511;3.64233 3.64233 3.64233 3.64233 3.64233 3.64233;3.65 3.65 3.65 3.65 3.65 3.65;3.65825 3.65825 3.65825 3.65825 3.65825 3.65825;3.6665 3.6665 3.6665 3.6665 3.6665 3.6665;3.67476 3.67476 3.67476 3.67476 3.67476 3.67476;3.68301 3.68301 3.68301 3.68301 3.68301 3.68301;3.69126 3.69126 3.69126 3.69126 3.69126 3.69126;3.69952 3.69952 3.69952 3.69952 3.69952 3.69952;3.70777 3.70777 3.70777 3.70777 3.70777 3.70777;3.71583 3.71583 3.71583 3.71583 3.71583 3.71583;3.72334 3.72334 3.72334 3.72334 3.72334 3.72334;3.73246 3.73246 3.73246 3.73246 3.73246 3.73246;3.74258 3.74258 3.74258 3.74258 3.74258 3.74258;3.75276 3.75276 3.75276 3.75276 3.75276 3.75276;3.76295 3.76295 3.76295 3.76295 3.76295 3.76295;3.77313 3.77313 3.77313 3.77313 3.77313 3.77313;3.78331 3.78331 3.78331 3.78331 3.78331 3.78331;3.7935 3.7935 3.7935 3.7935 3.7935 3.7935;3.80368 3.80368 3.80368 3.80368 3.80368 3.80368;3.81459 3.81459 3.81459 3.81459 3.81459 3.81459;3.82556 3.82556 3.82556 3.82556 3.82556 3.82556;3.83654 3.83654 3.83654 3.83654 3.83654 3.83654;3.84646 3.84646 3.84646 3.84646 3.84646 3.84646;3.85584 3.85584 3.85584 3.85584 3.85584 3.85584;3.86522 3.86522 3.86522 3.86522 3.86522 3.86522;3.87454 3.87454 3.87454 3.87454 3.87454 3.87454;3.8835 3.8835 3.8835 3.8835 3.8835 3.8835;3.89255 3.89255 3.89255 3.89255 3.89255 3.89255;3.9016 3.9016 3.9016 3.9016 3.9016 3.9016;3.91065 3.91065 3.91065 3.91065 3.91065 3.91065;3.91971 3.91971 3.91971 3.91971 3.91971 3.91971;3.92884 3.92884 3.92884 3.92884 3.92884 3.92884;3.93875 3.93875 3.93875 3.93875 3.93875 3.93875;3.95021 3.95021 3.95021 3.95021 3.95021 3.95021;3.96167 3.96167 3.96167 3.96167 3.96167 3.96167;3.97312 3.97312 3.97312 3.97312 3.97312 3.97312;3.98443 3.98443 3.98443 3.98443 3.98443 3.98443;3.99549 ...(+748 chars)] % Datasheet derived V  VoltageRange=[2.25 Inf] % Datasheet derived V  HysteresisModel=simscape.battery.enum.cells.HysteresisModel.none  MaximumHysteresisVoltage=[0, 0, 0, 0, 0, 0, 0] % Parameter not set V  InstantaneousHysteresisVoltage=[0, 0, 0, 0, 0, 0, 0] % Parameter not set V  HysteresisRate=0.1 % Parameter not set  MaximumHysteresisVoltageThermal=[0, 0, 0; 0, 0, 0; 0, 0, 0; 0, 0, 0; 0, 0, 0; 0, 0, 0; 0, 0, 0] % Parameter not set V  InstantaneousHysteresisVoltageThermal=[0, 0, 0; 0, 0, 0; 0, 0, 0; 0, 0, 0; 0, 0, 0; 0, 0, 0; 0, 0, 0] % Parameter not set V  HysteresisRateThermal=0.1 % Parameter not set  ResistanceSOCBreakpoints=[0 0.01 0.02 0.03 0.04 0.05 0.06 0.07 0.08 0.09 0.1 0.11 0.12 0.13 0.14 0.15 0.16 0.17 0.18 0.19 0.2 0.21 0.22 0.23 0.24 0.25 0.26 0.27 0.28 0.29 0.3 0.31 0.32 0.33 0.34 0.35 0.36 0.37 0.38 0.39 0.4 0.41 0.42 0.43 0.44 0.45 0.46 0.47 0.48 0.49 0.5 0.51 0.52 0.53 0.54 0.55 0.56 0.57 0.58 0.59 0.6 0.61 0.62 0.63 0.64 0.65 0.66 0.67 0.68 0.69 0.7 0.71 0.72 0.73 0.74 0.75 0.76 0.77 0.78 0.79 0.8 0.81 0.82 0.83 0.84 0.85 0.86 0.87 0.88 0.89 0.9 0.91 0.92 0.93 0.94 0.95 0.96 0.97 0.98 0.99 1] % Datasheet derived  ResistanceTemperatureBreakpoints=[-10 0 10 25 45 60] % Datasheet derived degC  ResistanceCurrentBreakpoints=[-1, 0, 1] % Parameter not set A  CurrentDependence=simscape.battery.enum.cells.CurrentDependence.Disabled  R0=[0.31638 0.3243 0.30647 0.2881 0.26534 0.23483 0.21466 0.1963 0.19065 0.18321 0.17517 0.17035 0.1686 0.16602 0.16263 0.16182 0.16098 0.16003 0.15908 0.15746 0.15485 0.15224 0.14963 0.14702 0.14441 0.14408 0.14309 0.14204 0.14098 0.13992 0.13886 0.13779 0.13673 0.13567 0.13461 0.13373 0.13328 0.13287 0.13246 0.13202 0.13158 0.13114 0.1307 0.13026 0.12982 0.12938 0.12894 0.12846 0.12829 0.12823 0.12821 0.1282 0.12818 0.12817 0.12815 0.12814 0.12812 0.12779 0.12659 0.12613 0.1261 0.12607 0.12605 0.12602 0.126 0.12598 0.12595 0.12709 0.12835 0.1296 0.13037 0.13088 0.1314 0.13182 0.13158 0.13136 0.13113 0.1309 0.13069 0.13059 0.13086 0.13184 0.13283 0.13381 0.13455 0.1349 0.13525 0.13561 0.13601 0.1363 0.13601 0.1347 0.13339 0.13211 0.13099 0.12903 0.12626 0.1235 0.12073 0.11181 0.10295] % Datasheet derived Ohm  R0I=[.0117, .0085, .009; .011, .0085, .009; .0114, .0087, .0092; .0107, .0082, .0088; .0107, .0083, .0091; .0113, .0085, .0089; .0116, .0085, .0089] % Parameter not set Ohm  R0Thermal=[1.5461 1.75516 2.11759 0.31638 0.46651 0.23498;1.5461 1.99954 2.27305 0.3243 0.34615 0.09965;1.5461 1.92281 2.1374 0.30647 0.20343 0.05211;1.5461 1.84609 2.00176 0.2881 0.15069 0.02648;1.5461 1.76937 1.86611 0.26534 0.12351 0.03545;1.5461 1.69264 1.73046 0.23483 0.10579 0.0319;1.5461 1.61592 1.59482 0.21466 0.09923 0.03983;1.5461 1.5392 1.45917 0.1963 0.0958 0.05105;1.5461 1.46247 1.32352 0.19065 0.10282 0.06344;1.5461 1.38575 1.18787 0.18321 0.10641 0.07241;1.5461 1.30902 1.05223 0.17517 0.10811 0.07828;1.5461 1.2323 0.91658 0.17035 0.11082 0.08499;1.5461 1.15558 0.78093 0.1686 0.11501 0.09321;1.50339 1.07885 0.64529 0.16602 0.11389 0.09611;1.46067 1.00213 0.52896 0.16263 0.11281 0.09693;1.41796 0.92541 0.45732 0.16182 0.1148 0.09886;1.37525 0.84868 0.40356 0.16098 0.11649 0.10041;1.33254 0.77196 0.35633 0.16003 0.1172 0.10099;1.28982 0.69523 0.32513 0.15908 0.11792 0.10158;1.24711 0.61749 0.29756 0.15746 0.11748 0.101;1.2044 0.5576 0.27681 0.15485 0.11475 0.09814;1.16169 0.50708 0.25953 0.15224 0.11202 0.09528;1.11897 0.46758 0.24304 0.14963 0.11054 0.09242;1.07626 0.43256 0.23145 0.14702 0.10939 0.09016;1.03355 0.40213 0.21986 0.14441 0.10825 0.08946;0.99084 0.37836 0.21479 0.14408 0.10821 0.08986;0.94812 0.35585 0.21092 0.14309 0.1066 0.08869;0.90541 0.33652 0.20677 0.14204 0.10481 0.08725;0.8627 0.32218 0.20275 0.14098 0.10391 0.08564;0.81999 0.30785 0.19912 0.13992 0.10301 0.08404;0.77727 0.29756 0.19549 0.13886 0.1021 0.08274;0.73457 0.28818 0.19186 0.13779 0.10125 0.08295;0.69186 0.2788 0.1889 0.13673 0.10088 0.08317;0.65043 0.27154 0.18649 0.13567 0.10051 0.08339;0.60913 0.26481 0.18408 0.13461 0.10013 0.0836;0.57538 0.25838 0.18198 0.13373 0.10007 0.08413;0.5481 0.25225 0.18022 0.13328 0.10029 0.08494;0.52084 0.24869 0.17996 0.13287 0.10054 0.08577;0.49467 0.24569 0.17968 0.13246 0.10076 0.08658;0.47265 0.24242 0.17912 0.13202 0.10071 0.08711;0.45063 0.23914 0.17856 0.13158 0.10065 0.08708;0.43278 0.23587 0.17801 0.13114 0.10056 0.08706;0.42113 0.23372 0.17745 0.1307 0.09993 0.08703;0.40948 0.23194 0.17689 0.13026 0.09931 0.087;0.39802 0.23016 0.17625 0.12982 0.09869 0.08698;0.3895 0.22838 0.17554 0.12938 0.09807 0.08695;0.38098 0.2266 0.17484 0.12894 0.09745 0.08692;0.37243 0.2248 0.17411 0.12846 0.09681 0.08688;0.36446 0.22399 0.17395 0.12829 0.09673 0.08739;0.35683 0.2238 0.17413 0.12823 0.097 0.08826;0.35467 0.22407 0.17478 0.12821 0.09771 0.08958;0.35251 0.22433 0.17543 0.1282 0.098 0.09079;0.35035 0.2246 0.17607 0.12818 0.09829 0.09028;0.34819 0.22487 0.17654 0.12817 0.09857 0.08977;0.34604 0.22513 0.17577 0.12815 0.09886 0.08925;0.34388 0.2254 0.175 0.12814 0.09915 0.08874;0.34172 0.22541 0.17423 0.12812 0.09944 0.08823;0.3394 0.22519 0.17331 0.12779 0.09957 0.08756;0.33667 0.22454 0.17196 0.12659 0.09928 0.08647;0.33518 0.22514 0.17187 0.12613 0.10014 0.08664;0.33524 0.22653 0.17256 0.1261 0.10082 0.08759;0.33556 0.22797 0.1733 0.12607 0.10155 0.0885;0.33589 0.22941 0.17405 0.12605 0.10227 0.08918;0.33622 0.23086 0.17484 0.12602 0.103 0.08985;0.33655 0.2323 0.1758 0.126 0.10373 0.09053;0.33688 0.23374 0.17676 0.12598 0.10446 0.0912;0.33721 0.23499 0.17772 0.12595 0.10519 0.09188;0.3381 0.23639 0.17924 0.12709 0.10648 0.09312;0.33905 0.23784 0.18082 0.12835 0.10783 0.09441;0.34 0.23929 0.18241 0.1296 0.10918 0.09571;0.34031 0.23991 0.18316 0.13037 0.1097 0.09618;0.34036 0.24011 0.18349 0.13088 0.1098 0.09608;0.3404 0.24031 0.18382 0.1314 0.10989 0.09597;0.3404 0.24047 0.1841 0.13182 0.10986 0.09581;0.34011 0.24033 0.1841 0.13158 0.10953 0.09535;0.33989 0.24027 0.18422 0.13136 0.10929 0.09498;0.34006 0.24021 0.18463 0.13113 0.10904 0.09461;0.34112 0.24015 0.18505 0.1309 0.1088 0.09423;0.34219 0.24057 0.18547 0.13069 0.10855 0.09385;0.34331 0.24158 0.18594 0.13059 0.10837 0.09322;0.34505 0.2432 0.18703 0.13086 0.10748 0.0932;0.348 0.24604 0.18933 0.13184 0.10774 0.09438;0.35095 0.24887 0.19163 0.13283 0.108 0.09557;0.35389 0.25171 0.19393 0.13381 0.10826 0.09676;0.35814 0.25442 0.19611 0.13455 0.1084 0.09783 ...(+755 chars)] % Datasheet derived Ohm  R0ThermalI=repmat([.0117, .0085, .009; .011, .0085, .009; .0114, .0087, .0092; .0107, .0082, .0088; .0107, .0083, .0091; .0113, .0085, .0089; .0116, .0085, .0089], 1, 1, 3) % Parameter not set Ohm  DischargeR0=[.0085, .0085, .0087, .0082, .0083, .0085, .0085] % Parameter not set Ohm  ChargeR0=[.0085, .0085, .0087, .0082, .0083, .0085, .0085] % Parameter not set Ohm  ChargeR0Thermal=[.0117, .0085, .009; .011, .0085, .009; .0114, .0087, .0092; .0107, .0082, .0088; .0107, .0083, .0091; .0113, .0085, .0089; .0116, .0085, .0089] % Parameter not set Ohm  DischargeR0Thermal=[.0117, .0085, .009; .011, .0085, .009; .0114, .0087, .0092; .0107, .0082, .0088; .0107, .0083, .0091; .0113, .0085, .0089; .0116, .0085, .0089] % Parameter not set Ohm  RCPairs=simscape.battery.enum.cells.RCPairs.noDynamics  R1=[.0029, .0024, .0026, .0016, .0023, .0018, .0017] % Parameter not set Ohm  Tau1=[36, 45, 105, 29, 77, 33, 39] % Parameter not set s  R2=[.0029, .0024, .0026, .0016, .0023, .0018, .0017] % Parameter not set Ohm  Tau2=[36, 45, 105, 29, 77, 33, 39] % Parameter not set s  R3=[.0029, .0024, .0026, .0016, .0023, .0018, .0017] % Parameter not set Ohm  Tau3=[36, 45, 105, 29, 77, 33, 39] % Parameter not set s  R1I=[.0109, .0029, .0013; .0069, .0024, .0012; .0047, .0026, .0013; .0034, .0016, .001; .0033, .0023, .0014; .0033, .0018, .0011; .0028, .0017, .0011] % Parameter not set Ohm  Tau1I=[20, 36, 39; 31, 45, 39; 109, 105, 61; 36, 29, 26; 59, 77, 67; 40, 33, 29; 25, 39, 33] % Parameter not set s  R2I=[.0109, .0029, .0013; .0069, .0024, .0012; .0047, .0026, .0013; .0034, .0016, .001; .0033, .0023, .0014; .0033, .0018, .0011; .0028, .0017, .0011] % Parameter not set Ohm  Tau2I=[20, 36, 39; 31, 45, 39; 109, 105, 61; 36, 29, 26; 59, 77, 67; 40, 33, 29; 25, 39, 33] % Parameter not set s  R3I=[.0109, .0029, .0013; .0069, .0024, .0012; .0047, .0026, .0013; .0034, .0016, .001; .0033, .0023, .0014; .0033, .0018, .0011; .0028, .0017, .0011] % Parameter not set Ohm  Tau3I=[20, 36, 39; 31, 45, 39; 109, 105, 61; 36, 29, 26; 59, 77, 67; 40, 33, 29; 25, 39, 33] % Parameter not set s  DischargeR1=[.0029, .0024, .0026, .0016, .0023, .0018, .0017] % Parameter not set Ohm  DischargeTau1=[36, 45, 105, 29, 77, 33, 39] % Parameter not set s  ChargeR1=[.0029, .0024, .0026, .0016, .0023, .0018, .0017] % Parameter not set Ohm  ChargeTau1=[36, 45, 105, 29, 77, 33, 39] % Parameter not set s  DischargeR2=[.0029, .0024, .0026, .0016, .0023, .0018, .0017] % Parameter not set Ohm  DischargeTau2=[36, 45, 105, 29, 77, 33, 39] % Parameter not set s  ChargeR2=[.0029, .0024, .0026, .0016, .0023, .0018, .0017] % Parameter not set Ohm  ChargeTau2=[36, 45, 105, 29, 77, 33, 39] % Parameter not set s  DischargeR3=[.0029, .0024, .0026, .0016, .0023, .0018, .0017] % Parameter not set Ohm  DischargeTau3=[36, 45, 105, 29, 77, 33, 39] % Parameter not set s  ChargeR3=[.0029, .0024, .0026, .0016, .0023, .0018, .0017] % Parameter not set Ohm  ChargeTau3=[36, 45, 105, 29, 77, 33, 39] % Parameter not set s  R1Thermal=[.0109, .0029, .0013; .0069, .0024, .0012; .0047, .0026, .0013; .0034, .0016, .001; .0033, .0023, .0014; .0033, .0018, .0011; .0028, .0017, .0011] % Parameter not set Ohm  Tau1Thermal=[20, 36, 39; 31, 45, 39; 109, 105, 61; 36, 29, 26; 59, 77, 67; 40, 33, 29; 25, 39, 33] % Parameter not set s  R2Thermal=[.0109, .0029, .0013; .0069, .0024, .0012; .0047, .0026, .0013; .0034, .0016, .001; .0033, .0023, .0014; .0033, .0018, .0011; .0028, .0017, .0011] % Parameter not set Ohm  Tau2Thermal=[20, 36, 39; 31, 45, 39; 109, 105, 61; 36, 29, 26; 59, 77, 67; 40, 33, 29; 25, 39, 33] % Parameter not set s  R3Thermal=[.0109, .0029, .0013; .0069, .0024, .0012; .0047, .0026, .0013; .0034, .0016, .001; .0033, .0023, .0014; .0033, .0018, .0011; .0028, .0017, .0011] % Parameter not set Ohm  Tau3Thermal=[20, 36, 39; 31, 45, 39; 109, 105, 61; 36, 29, 26; 59, 77, 67; 40, 33, 29; 25, 39, 33] % Parameter not set s  R1ThermalI=repmat([.0109, .0029, .0013; .0069, .0024, .0012; .0047, .0026, .0013; .0034, .0016, .001; .0033, .0023, .0014; .0033, .0018, .0011; .0028, .0017, .0011], 1, 1, 3) % Parameter not set Ohm  Tau1ThermalI=repmat([20, 36, 39; 31, 45, 39; 109, 105, 61; 36, 29, 26; 59, 77, 67; 40, 33, 29; 25, 39, 33], 1, 1, 3) % Parameter not set s  R2ThermalI=repmat([.0109, .0029, .0013; .0069, .0024, .0012; .0047, .0026, .0013; .0034, .0016, .001; .0033, .0023, .0014; .0033, .0018, .0011; .0028, .0017, .0011], 1, 1, 3) % Parameter not set Ohm  Tau2ThermalI=repmat([20, 36, 39; 31, 45, 39; 109, 105, 61; 36, 29, 26; 59, 77, 67; 40, 33, 29; 25, 39, 33], 1, 1, 3) % Parameter not set s  R3ThermalI=repmat([.0109, .0029, .0013; .0069, .0024, .0012; .0047, .0026, .0013; .0034, .0016, .001; .0033, .0023, .0014; .0033, .0018, .0011; .0028, .0017, .0011], 1, 1, 3) % Parameter not set Ohm  Tau3ThermalI=repmat([20, 36, 39; 31, 45, 39; 109, 105, 61; 36, 29, 26; 59, 77, 67; 40, 33, 29; 25, 39, 33], 1, 1, 3) % Parameter not set s  DischargeR1Thermal=[.0109, .0029, .0013; .0069, .0024, .0012; .0047, .0026, .0013; .0034, .0016, .001; .0033, .0023, .0014; .0033, .0018, .0011; .0028, .0017, .0011] % Parameter not set Ohm  DischargeTau1Thermal=[20, 36, 39; 31, 45, 39; 109, 105, 61; 36, 29, 26; 59, 77, 67; 40, 33, 29; 25, 39, 33] % Parameter not set s  ChargeR1Thermal=[.0109, .0029, .0013; .0069, .0024, .0012; .0047, .0026, .0013; .0034, .0016, .001; .0033, .0023, .0014; .0033, .0018, .0011; .0028, .0017, .0011] % Parameter not set Ohm  ChargeTau1Thermal=[20, 36, 39; 31, 45, 39; 109, 105, 61; 36, 29, 26; 59, 77, 67; 40, 33, 29; 25, 39, 33] % Parameter not set s  DischargeR2Thermal=[.0109, .0029, .0013; .0069, .0024, .0012; .0047, .0026, .0013; .0034, .0016, .001; .0033, .0023, .0014; .0033, .0018, .0011; .0028, .0017, .0011] % Parameter not set Ohm  DischargeTau2Thermal=[20, 36, 39; 31, 45, 39; 109, 105, 61; 36, 29, 26; 59, 77, 67; 40, 33, 29; 25, 39, 33] % Parameter not set s  ChargeR2Thermal=[.0109, .0029, .0013; .0069, .0024, .0012; .0047, .0026, .0013; .0034, .0016, .001; .0033, .0023, .0014; .0033, .0018, .0011; .0028, .0017, .0011] % Parameter not set Ohm  ChargeTau2Thermal=[20, 36, 39; 31, 45, 39; 109, 105, 61; 36, 29, 26; 59, 77, 67; 40, 33, 29; 25, 39, 33] % Parameter not set s  DischargeR3Thermal=[.0109, .0029, .0013; .0069, .0024, .0012; .0047, .0026, .0013; .0034, .0016, .001; .0033, .0023, .0014; .0033, .0018, .0011; .0028, .0017, .0011] % Parameter not set Ohm  DischargeTau3Thermal=[20, 36, 39; 31, 45, 39; 109, 105, 61; 36, 29, 26; 59, 77, 67; 40, 33, 29; 25, 39, 33] % Parameter not set s  ChargeR3Thermal=[.0109, .0029, .0013; .0069, .0024, .0012; .0047, .0026, .0013; .0034, .0016, .001; .0033, .0023, .0014; .0033, .0018, .0011; .0028, .0017, .0011] % Parameter not set Ohm  ChargeTau3Thermal=[20, 36, 39; 31, 45, 39; 109, 105, 61; 36, 29, 26; 59, 77, 67; 40, 33, 29; 25, 39, 33] % Parameter not set s  SelfDischargeResistor=simscape.battery.enum.cells.BatteryEnable.Disabled  SelfDischargeR=7e3 % Parameter not set Ohm  SelfDischargeRThermal=[8000, 7000, 6000] % Parameter not set Ohm  CyclingAgingMethod=simscape.battery.enum.cells.CyclingAgingMethod.tableN  CycleCalculationMethod=simscape.battery.enum.cells.CycleCalculationMethod.EquivalentCycles  NumDisCycles=100 % Parameter not set  OCVChange=0 % Parameter not set  R0Change=0 % Parameter not set  CapacityChange=0 % Parameter not set  SelfDischargeRChange=0 % Parameter not set  R1Change=0 % Parameter not set  R2Change=0 % Parameter not set  R3Change=0 % Parameter not set  NumDisCyclesBreakpoints=[0 7 13 19 25 31 37 43 49 55 61 67 73 79 85 91 97 103 109 115 121 127 133 139 145 151 157 163 169 175 181 187 193 199 205 211 217 223 229 235 241 247 253 259 265 271 277 283 289 295 301 307 313 319 325 331 337 343 349 355 361 367 373 379 385 391 397 403 409 415 421 427 433 439 445 451 457 463 469 475 481 487 493 499] % Datasheet derived  AgingTemperatureBreakpoints=[298.15, 323.15] % Parameter not set K  AgingCurrentBreakpoints=[-.1, -.5, -5] % Parameter not set A  OCVChangeVec=[0 -0.2056 -0.4112 -0.602 -0.7529 -0.9041 -1.0234 -1.116 -1.2087 -1.3013 -1.3939 -1.4865 -1.5404 -1.5936 -1.6468 -1.7 -1.7534 -1.807 -1.8607 -1.9143 -1.972 -2.0316 -2.0912 -2.1507 -2.2103 -2.2687 -2.3264 -2.3842 -2.442 -2.4996 -2.5474 -2.5914 -2.6354 -2.6795 -2.7235 -2.7676 -2.8116 -2.8556 -2.8997 -2.9437 -2.9899 -3.057 -3.1273 -3.1975 -3.2718 -3.347 -3.4222 -3.4977 -3.5744 -3.6428 -3.6945 -3.7461 -3.7966 -3.8466 -3.8965 -3.9465 -3.9964 -4.0461 -4.0951 -4.1498 -4.2072 -4.2646 -4.322 -4.3794 -4.4368 -4.4942 -4.5515 -4.61 -4.6685 -4.7269 -4.7854 -4.844 -4.9032 -4.9624 -5.0216 -5.0808 -5.1413 -5.2041 -5.2668 -5.3295 -5.3922 -5.455 -5.5177 -5.5804] % Datasheet derived  OCVChangeThermal=[0, 0; 0, 0; 0, 0; 0, 0] % Parameter not set  R0ChangeVec=[0 0 0 0 0 0 0 0 0 0 0 0 0 0 0 0 0 0 0 0 0 0 0 0 0 0 0 0 0 0 0 0 0 0 0 0 0 0 0 0 0 0 0 0 0 0 0 0 0 0 0 0 0 0 0 0 0 0 0 0 0 0 0 0 0 0 0 0 0 0 0 0 0 0 0 0 0 0 0 0 0 0 0 0] % Parameter assumed  R0ChangeThermal=[0, 0; 0, 0; 0, 0; 0, 0] % Parameter not set  R0ChangeThermalI=repmat(0, 4, 2, 3) % Parameter not set  R0CyclingChangeInitialTarget=0 % Parameter not set  CapacityChangeVec=[0 -0.367 -0.733 -1.1 -1.466 -1.834 -2.202 -2.571 -2.94 -3.309 -3.678 -4.047 -4.261 -4.473 -4.685 -4.897 -5.109 -5.32 -5.532 -5.744 -5.972 -6.21 -6.448 -6.686 -6.924 -7.162 -7.4 -7.638 -7.876 -8.114 -8.313 -8.496 -8.679 -8.862 -9.045 -9.228 -9.411 -9.593 -9.776 -9.959 -10.142 -10.405 -10.679 -10.954 -11.228 -11.503 -11.777 -12.052 -12.326 -12.571 -12.756 -12.941 -13.126 -13.311 -13.496 -13.681 -13.866 -14.051 -14.235 -14.442 -14.659 -14.875 -15.092 -15.308 -15.525 -15.741 -15.958 -16.175 -16.391 -16.607 -16.822 -17.038 -17.254 -17.47 -17.685 -17.901 -18.122 -18.35 -18.579 -18.807 -19.036 -19.265 -19.493 -19.722] % Datasheet derived  CapacityChangeThermal=[0, 0; 0, 0; 0, 0; 0, 0] % Parameter not set  CapacityChangeThermalI=repmat(0, 4, 2, 3) % Parameter not set  CapacityCyclingChangeInitialTarget=0 % Parameter not set  SelfDischargeRChangeVec=[0, 0, 0, 0] % Parameter not set  SelfDischargeRChangeThermal=[0, 0; 0, 0; 0, 0; 0, 0] % Parameter not set  SelfDischargeRChangeThermalI=repmat(0, 4, 2, 3) % Parameter not set  SelfDischargeRCyclingChangeInitialTarget=0 % Parameter not set  R1ChangeVec=[0, 0, 0, 0] % Parameter not set  R1ChangeThermal=[0, 0; 0, 0; 0, 0; 0, 0] % Parameter not set  R1ChangeThermalI=repmat(0, 4, 2, 3) % Parameter not set  R1CyclingChangeInitialTarget=0 % Parameter not set  R2ChangeVec=[0, 0, 0, 0] % Parameter not set  R2ChangeThermal=[0, 0; 0, 0; 0, 0; 0, 0] % Parameter not set  R2ChangeThermalI=repmat(0, 4, 2, 3) % Parameter not set  R2CyclingChangeInitialTarget=0 % Parameter not set  R3ChangeVec=[0, 0, 0, 0] % Parameter not set  R3ChangeThermal=[0, 0; 0, 0; 0, 0; 0, 0] % Parameter not set  R3ChangeThermalI=repmat(0, 4, 2, 3) % Parameter not set  R3CyclingChangeInitialTarget=0 % Parameter not set  CalendarAgeResistance=simscape.battery.enum.cells.BatteryEnable.Disabled  CalendarAgeCapacity=simscape.battery.enum.cells.BatteryEnable.Disabled  CalendarAgingMethod=simscape.battery.enum.cells.CalendarAgingMethod.equation  StorageVariable=simscape.battery.enum.cells.StorageVariable.OCV  OCVDuringStorage=0.9 % Parameter not set  SOCDuringStorage=0.6 % Parameter not set  StorageTimeIntervals=[0] % Parameter not set d  StorageTemperatures=[273] % Parameter not set K  ResistanceScalingOCV=2.2134e6 % Parameter not set  ResistanceScalingOCVOffset=1.632e6 % Parameter not set  ResistanceExponentialIncrease=0.515833569 % Parameter not set V  ResistanceTimeExponent=0.75 % Parameter not set  ResistanceAgeTemperatureBreakpoints=[273.15, 298.15, 323.15] % Parameter not set K  ResistanceAgeTimeBreakpoints=[0, 90, 180, 270] % Parameter not set d  PercentResistanceChange=[0, 0, 0] % Parameter not set  ResistanceTimeBreakpoints=100 % Parameter not set d  PercentResistanceChangeThermal=[0, 0, 0; 0, 0, 0; 0, 0, 0; 0, 0, 0] % Parameter not set  CapacityScalingOCV=1.5097e07 % Parameter not set  CapacityScalingOCVOffset=8.3625e06 % Parameter not set  CapacityExponentialIncrease=0.6011 % Parameter not set V  CapacityTimeExponent=0.75 % Parameter not set  CapacityAgeTemperatureBreakpoints=[273.15, 298.15, 323.15] % Parameter not set K  CapacityAgeTimeBreakpoints=[0, 90, 180, 270] % Parameter not set d  PercentCapacityChange=[0, 0, 0] % Parameter not set  CapacityTimeBreakpoints=100 % Parameter not set d  PercentCapacityChangeThermal=[0, 0, 0; 0, 0, 0; 0, 0, 0; 0, 0, 0] % Parameter not set  SimulationTemperature=298.15 % Parameter not set K  BatteryThermalMass=20.7 % Parameter assumed J/K  NumThermalModels=6 % Parameter not set  ThermalConductivityZ=18 % Parameter not set W/(K*m)  CrossSectionalAreaXY=0.000286 m^2  Height=0.036 m  ReversibleHeatModel=simscape.battery.enum.cells.ReversibleHeatModel.Disabled  EntropicCoefficient=[0, 0, 0, 0, 0, 0, 0] % Parameter not set mV/K  CurrentDirectionality=simscape.battery.enum.cells.BatteryEnable.Disabled  stateOfCharge_specify=off  stateOfCharge_priority=High  stateOfCharge=1  stateOfCharge_nominal_specify=off  stateOfCharge_nominal_value=1  stateOfCharge_nominal_unit=1  batteryVoltage_specify=off  batteryVoltage_priority=None  batteryVoltage=0 V  batteryVoltage_nominal_specify=off  batteryVoltage_nominal_value=1  batteryVoltage_nominal_unit=V  batteryCurrent_specify=off  batteryCurrent_priority=None  batteryCurrent=0 A  batteryCurrent_nominal_specify=off  batteryCurrent_nominal_value=1  batteryCurrent_nominal_unit=A  numCycles_specify=off  numCycles_priority=High  numCycles=0  numCycles_nominal_specify=off  numCycles_nominal_value=1  numCycles_nominal_unit=1  batteryTemperature_specify=off  batteryTemperature_priority=High  batteryTemperature=298.15 K  batteryTemperature_nominal_specify=off  batteryTemperature_nominal_value=1  batteryTemperature_nominal_unit=K  hysteresisState_specify=off  hysteresisState_priority=High  hysteresisState=0  hysteresisState_nominal_specify=off  hysteresisState_nominal_value=1  hysteresisState_nominal_unit=1  isExothermFaulted_specify=off  isExothermFaulted_priority=None  isExothermFaulted=0  isExothermFaulted_nominal_specify=off  isExothermFaulted_nominal_value=1  isExothermFaulted_nominal_unit=1  reactionHeatRate_specify=off  reactionHeatRate_priority=None  reactionHeatRate=0 W  reactionHeatRate_nominal_specify=off  reactionHeatRate_nominal_value=1  reactionHeatRate_nominal_unit=W  reactionExtent_specify=off  reactionExtent_priority=None  reactionExtent=0  reactionExtent_nominal_specify=off  reactionExtent_nominal_value=1  reactionExtent_nominal_unit=1
      settings: AttributesFormatString=Panasonic:NCA843436  InternalSimscapePortConfiguration="{\"Bottom\":[{\"id\":\"n\",\"label\":\"-\",\"type\":\"foundation.electrical.electrical\"},{\"id\":\"H\",\"label\":\"H\",\"type\":\"foundation.thermal.thermal\"}],\"Left\":[],\"Right\":[],\"Top\":[{\"id\":\"p\",\"label\":\"+\",\"type\":\"foundation.electrical.electrical\"}]}"
  Battery Equivalent Circuit4 : batt_lib/Cells/Battery Equivalent Circuit  PartSpecification="{\"CollectionId\":\"SimscapeBattery\",\"CollectionVersion\":\"1.0.0\",\"DatasetId\":\"Panasonic|NCA843436|simscape.battery.batteryEquivalentCircuit\",\"DisplayName\":\"Panasonic:NCA843436\"}"  BatteryCapacity=1.354 % Datasheet derived hr*A  ThermalModel=simscape.battery.enum.cells.BatteryThermalModel.LumpedThermalMass  ExtrapolationMethod=simscape.enum.extrapolation.linear  SOCBreakpoints=[0 0.01 0.02 0.03 0.04 0.05 0.06 0.07 0.08 0.09 0.1 0.11 0.12 0.13 0.14 0.15 0.16 0.17 0.18 0.19 0.2 0.21 0.22 0.23 0.24 0.25 0.26 0.27 0.28 0.29 0.3 0.31 0.32 0.33 0.34 0.35 0.36 0.37 0.38 0.39 0.4 0.41 0.42 0.43 0.44 0.45 0.46 0.47 0.48 0.49 0.5 0.51 0.52 0.53 0.54 0.55 0.56 0.57 0.58 0.59 0.6 0.61 0.62 0.63 0.64 0.65 0.66 0.67 0.68 0.69 0.7 0.71 0.72 0.73 0.74 0.75 0.76 0.77 0.78 0.79 0.8 0.81 0.82 0.83 0.84 0.85 0.86 0.87 0.88 0.89 0.9 0.91 0.92 0.93 0.94 0.95 0.96 0.97 0.98 0.99 1] % Datasheet derived  TemperatureBreakpoints=[-10 0 10 25 45 60] % Datasheet derived degC  OpenCircuitVoltage=[2.817 2.94537 3.0182 3.08984 3.15197 3.18868 3.22389 3.25188 3.27953 3.3028 3.32214 3.34136 3.36247 3.37682 3.38851 3.4018 3.4147 3.42636 3.43803 3.44822 3.45549 3.46277 3.47005 3.47732 3.4846 3.49328 3.49997 3.50631 3.51243 3.51855 3.52468 3.5308 3.53692 3.54304 3.54917 3.55568 3.56257 3.56948 3.57636 3.58289 3.58942 3.59595 3.60248 3.60901 3.61554 3.62207 3.62861 3.63511 3.64233 3.65 3.65825 3.6665 3.67476 3.68301 3.69126 3.69952 3.70777 3.71583 3.72334 3.73246 3.74258 3.75276 3.76295 3.77313 3.78331 3.7935 3.80368 3.81459 3.82556 3.83654 3.84646 3.85584 3.86522 3.87454 3.8835 3.89255 3.9016 3.91065 3.91971 3.92884 3.93875 3.95021 3.96167 3.97312 3.98443 3.99549 4.00655 4.01783 4.0295 4.04093 4.05161 4.06166 4.07171 4.08185 4.09229 4.10286 4.11335 4.12383 4.13431 4.1515 4.17492] % Datasheet derived V  OpenCircuitVoltageThermal=[2.817 2.817 2.817 2.817 2.817 2.817;2.94537 2.94537 2.94537 2.94537 2.94537 2.94537;3.0182 3.0182 3.0182 3.0182 3.0182 3.0182;3.08984 3.08984 3.08984 3.08984 3.08984 3.08984;3.15197 3.15197 3.15197 3.15197 3.15197 3.15197;3.18868 3.18868 3.18868 3.18868 3.18868 3.18868;3.22389 3.22389 3.22389 3.22389 3.22389 3.22389;3.25188 3.25188 3.25188 3.25188 3.25188 3.25188;3.27953 3.27953 3.27953 3.27953 3.27953 3.27953;3.3028 3.3028 3.3028 3.3028 3.3028 3.3028;3.32214 3.32214 3.32214 3.32214 3.32214 3.32214;3.34136 3.34136 3.34136 3.34136 3.34136 3.34136;3.36247 3.36247 3.36247 3.36247 3.36247 3.36247;3.37682 3.37682 3.37682 3.37682 3.37682 3.37682;3.38851 3.38851 3.38851 3.38851 3.38851 3.38851;3.4018 3.4018 3.4018 3.4018 3.4018 3.4018;3.4147 3.4147 3.4147 3.4147 3.4147 3.4147;3.42636 3.42636 3.42636 3.42636 3.42636 3.42636;3.43803 3.43803 3.43803 3.43803 3.43803 3.43803;3.44822 3.44822 3.44822 3.44822 3.44822 3.44822;3.45549 3.45549 3.45549 3.45549 3.45549 3.45549;3.46277 3.46277 3.46277 3.46277 3.46277 3.46277;3.47005 3.47005 3.47005 3.47005 3.47005 3.47005;3.47732 3.47732 3.47732 3.47732 3.47732 3.47732;3.4846 3.4846 3.4846 3.4846 3.4846 3.4846;3.49328 3.49328 3.49328 3.49328 3.49328 3.49328;3.49997 3.49997 3.49997 3.49997 3.49997 3.49997;3.50631 3.50631 3.50631 3.50631 3.50631 3.50631;3.51243 3.51243 3.51243 3.51243 3.51243 3.51243;3.51855 3.51855 3.51855 3.51855 3.51855 3.51855;3.52468 3.52468 3.52468 3.52468 3.52468 3.52468;3.5308 3.5308 3.5308 3.5308 3.5308 3.5308;3.53692 3.53692 3.53692 3.53692 3.53692 3.53692;3.54304 3.54304 3.54304 3.54304 3.54304 3.54304;3.54917 3.54917 3.54917 3.54917 3.54917 3.54917;3.55568 3.55568 3.55568 3.55568 3.55568 3.55568;3.56257 3.56257 3.56257 3.56257 3.56257 3.56257;3.56948 3.56948 3.56948 3.56948 3.56948 3.56948;3.57636 3.57636 3.57636 3.57636 3.57636 3.57636;3.58289 3.58289 3.58289 3.58289 3.58289 3.58289;3.58942 3.58942 3.58942 3.58942 3.58942 3.58942;3.59595 3.59595 3.59595 3.59595 3.59595 3.59595;3.60248 3.60248 3.60248 3.60248 3.60248 3.60248;3.60901 3.60901 3.60901 3.60901 3.60901 3.60901;3.61554 3.61554 3.61554 3.61554 3.61554 3.61554;3.62207 3.62207 3.62207 3.62207 3.62207 3.62207;3.62861 3.62861 3.62861 3.62861 3.62861 3.62861;3.63511 3.63511 3.63511 3.63511 3.63511 3.63511;3.64233 3.64233 3.64233 3.64233 3.64233 3.64233;3.65 3.65 3.65 3.65 3.65 3.65;3.65825 3.65825 3.65825 3.65825 3.65825 3.65825;3.6665 3.6665 3.6665 3.6665 3.6665 3.6665;3.67476 3.67476 3.67476 3.67476 3.67476 3.67476;3.68301 3.68301 3.68301 3.68301 3.68301 3.68301;3.69126 3.69126 3.69126 3.69126 3.69126 3.69126;3.69952 3.69952 3.69952 3.69952 3.69952 3.69952;3.70777 3.70777 3.70777 3.70777 3.70777 3.70777;3.71583 3.71583 3.71583 3.71583 3.71583 3.71583;3.72334 3.72334 3.72334 3.72334 3.72334 3.72334;3.73246 3.73246 3.73246 3.73246 3.73246 3.73246;3.74258 3.74258 3.74258 3.74258 3.74258 3.74258;3.75276 3.75276 3.75276 3.75276 3.75276 3.75276;3.76295 3.76295 3.76295 3.76295 3.76295 3.76295;3.77313 3.77313 3.77313 3.77313 3.77313 3.77313;3.78331 3.78331 3.78331 3.78331 3.78331 3.78331;3.7935 3.7935 3.7935 3.7935 3.7935 3.7935;3.80368 3.80368 3.80368 3.80368 3.80368 3.80368;3.81459 3.81459 3.81459 3.81459 3.81459 3.81459;3.82556 3.82556 3.82556 3.82556 3.82556 3.82556;3.83654 3.83654 3.83654 3.83654 3.83654 3.83654;3.84646 3.84646 3.84646 3.84646 3.84646 3.84646;3.85584 3.85584 3.85584 3.85584 3.85584 3.85584;3.86522 3.86522 3.86522 3.86522 3.86522 3.86522;3.87454 3.87454 3.87454 3.87454 3.87454 3.87454;3.8835 3.8835 3.8835 3.8835 3.8835 3.8835;3.89255 3.89255 3.89255 3.89255 3.89255 3.89255;3.9016 3.9016 3.9016 3.9016 3.9016 3.9016;3.91065 3.91065 3.91065 3.91065 3.91065 3.91065;3.91971 3.91971 3.91971 3.91971 3.91971 3.91971;3.92884 3.92884 3.92884 3.92884 3.92884 3.92884;3.93875 3.93875 3.93875 3.93875 3.93875 3.93875;3.95021 3.95021 3.95021 3.95021 3.95021 3.95021;3.96167 3.96167 3.96167 3.96167 3.96167 3.96167;3.97312 3.97312 3.97312 3.97312 3.97312 3.97312;3.98443 3.98443 3.98443 3.98443 3.98443 3.98443;3.99549 ...(+748 chars)] % Datasheet derived V  VoltageRange=[2.25 Inf] % Datasheet derived V  HysteresisModel=simscape.battery.enum.cells.HysteresisModel.none  MaximumHysteresisVoltage=[0, 0, 0, 0, 0, 0, 0] % Parameter not set V  InstantaneousHysteresisVoltage=[0, 0, 0, 0, 0, 0, 0] % Parameter not set V  HysteresisRate=0.1 % Parameter not set  MaximumHysteresisVoltageThermal=[0, 0, 0; 0, 0, 0; 0, 0, 0; 0, 0, 0; 0, 0, 0; 0, 0, 0; 0, 0, 0] % Parameter not set V  InstantaneousHysteresisVoltageThermal=[0, 0, 0; 0, 0, 0; 0, 0, 0; 0, 0, 0; 0, 0, 0; 0, 0, 0; 0, 0, 0] % Parameter not set V  HysteresisRateThermal=0.1 % Parameter not set  ResistanceSOCBreakpoints=[0 0.01 0.02 0.03 0.04 0.05 0.06 0.07 0.08 0.09 0.1 0.11 0.12 0.13 0.14 0.15 0.16 0.17 0.18 0.19 0.2 0.21 0.22 0.23 0.24 0.25 0.26 0.27 0.28 0.29 0.3 0.31 0.32 0.33 0.34 0.35 0.36 0.37 0.38 0.39 0.4 0.41 0.42 0.43 0.44 0.45 0.46 0.47 0.48 0.49 0.5 0.51 0.52 0.53 0.54 0.55 0.56 0.57 0.58 0.59 0.6 0.61 0.62 0.63 0.64 0.65 0.66 0.67 0.68 0.69 0.7 0.71 0.72 0.73 0.74 0.75 0.76 0.77 0.78 0.79 0.8 0.81 0.82 0.83 0.84 0.85 0.86 0.87 0.88 0.89 0.9 0.91 0.92 0.93 0.94 0.95 0.96 0.97 0.98 0.99 1] % Datasheet derived  ResistanceTemperatureBreakpoints=[-10 0 10 25 45 60] % Datasheet derived degC  ResistanceCurrentBreakpoints=[-1, 0, 1] % Parameter not set A  CurrentDependence=simscape.battery.enum.cells.CurrentDependence.Disabled  R0=[0.31638 0.3243 0.30647 0.2881 0.26534 0.23483 0.21466 0.1963 0.19065 0.18321 0.17517 0.17035 0.1686 0.16602 0.16263 0.16182 0.16098 0.16003 0.15908 0.15746 0.15485 0.15224 0.14963 0.14702 0.14441 0.14408 0.14309 0.14204 0.14098 0.13992 0.13886 0.13779 0.13673 0.13567 0.13461 0.13373 0.13328 0.13287 0.13246 0.13202 0.13158 0.13114 0.1307 0.13026 0.12982 0.12938 0.12894 0.12846 0.12829 0.12823 0.12821 0.1282 0.12818 0.12817 0.12815 0.12814 0.12812 0.12779 0.12659 0.12613 0.1261 0.12607 0.12605 0.12602 0.126 0.12598 0.12595 0.12709 0.12835 0.1296 0.13037 0.13088 0.1314 0.13182 0.13158 0.13136 0.13113 0.1309 0.13069 0.13059 0.13086 0.13184 0.13283 0.13381 0.13455 0.1349 0.13525 0.13561 0.13601 0.1363 0.13601 0.1347 0.13339 0.13211 0.13099 0.12903 0.12626 0.1235 0.12073 0.11181 0.10295] % Datasheet derived Ohm  R0I=[.0117, .0085, .009; .011, .0085, .009; .0114, .0087, .0092; .0107, .0082, .0088; .0107, .0083, .0091; .0113, .0085, .0089; .0116, .0085, .0089] % Parameter not set Ohm  R0Thermal=[1.5461 1.75516 2.11759 0.31638 0.46651 0.23498;1.5461 1.99954 2.27305 0.3243 0.34615 0.09965;1.5461 1.92281 2.1374 0.30647 0.20343 0.05211;1.5461 1.84609 2.00176 0.2881 0.15069 0.02648;1.5461 1.76937 1.86611 0.26534 0.12351 0.03545;1.5461 1.69264 1.73046 0.23483 0.10579 0.0319;1.5461 1.61592 1.59482 0.21466 0.09923 0.03983;1.5461 1.5392 1.45917 0.1963 0.0958 0.05105;1.5461 1.46247 1.32352 0.19065 0.10282 0.06344;1.5461 1.38575 1.18787 0.18321 0.10641 0.07241;1.5461 1.30902 1.05223 0.17517 0.10811 0.07828;1.5461 1.2323 0.91658 0.17035 0.11082 0.08499;1.5461 1.15558 0.78093 0.1686 0.11501 0.09321;1.50339 1.07885 0.64529 0.16602 0.11389 0.09611;1.46067 1.00213 0.52896 0.16263 0.11281 0.09693;1.41796 0.92541 0.45732 0.16182 0.1148 0.09886;1.37525 0.84868 0.40356 0.16098 0.11649 0.10041;1.33254 0.77196 0.35633 0.16003 0.1172 0.10099;1.28982 0.69523 0.32513 0.15908 0.11792 0.10158;1.24711 0.61749 0.29756 0.15746 0.11748 0.101;1.2044 0.5576 0.27681 0.15485 0.11475 0.09814;1.16169 0.50708 0.25953 0.15224 0.11202 0.09528;1.11897 0.46758 0.24304 0.14963 0.11054 0.09242;1.07626 0.43256 0.23145 0.14702 0.10939 0.09016;1.03355 0.40213 0.21986 0.14441 0.10825 0.08946;0.99084 0.37836 0.21479 0.14408 0.10821 0.08986;0.94812 0.35585 0.21092 0.14309 0.1066 0.08869;0.90541 0.33652 0.20677 0.14204 0.10481 0.08725;0.8627 0.32218 0.20275 0.14098 0.10391 0.08564;0.81999 0.30785 0.19912 0.13992 0.10301 0.08404;0.77727 0.29756 0.19549 0.13886 0.1021 0.08274;0.73457 0.28818 0.19186 0.13779 0.10125 0.08295;0.69186 0.2788 0.1889 0.13673 0.10088 0.08317;0.65043 0.27154 0.18649 0.13567 0.10051 0.08339;0.60913 0.26481 0.18408 0.13461 0.10013 0.0836;0.57538 0.25838 0.18198 0.13373 0.10007 0.08413;0.5481 0.25225 0.18022 0.13328 0.10029 0.08494;0.52084 0.24869 0.17996 0.13287 0.10054 0.08577;0.49467 0.24569 0.17968 0.13246 0.10076 0.08658;0.47265 0.24242 0.17912 0.13202 0.10071 0.08711;0.45063 0.23914 0.17856 0.13158 0.10065 0.08708;0.43278 0.23587 0.17801 0.13114 0.10056 0.08706;0.42113 0.23372 0.17745 0.1307 0.09993 0.08703;0.40948 0.23194 0.17689 0.13026 0.09931 0.087;0.39802 0.23016 0.17625 0.12982 0.09869 0.08698;0.3895 0.22838 0.17554 0.12938 0.09807 0.08695;0.38098 0.2266 0.17484 0.12894 0.09745 0.08692;0.37243 0.2248 0.17411 0.12846 0.09681 0.08688;0.36446 0.22399 0.17395 0.12829 0.09673 0.08739;0.35683 0.2238 0.17413 0.12823 0.097 0.08826;0.35467 0.22407 0.17478 0.12821 0.09771 0.08958;0.35251 0.22433 0.17543 0.1282 0.098 0.09079;0.35035 0.2246 0.17607 0.12818 0.09829 0.09028;0.34819 0.22487 0.17654 0.12817 0.09857 0.08977;0.34604 0.22513 0.17577 0.12815 0.09886 0.08925;0.34388 0.2254 0.175 0.12814 0.09915 0.08874;0.34172 0.22541 0.17423 0.12812 0.09944 0.08823;0.3394 0.22519 0.17331 0.12779 0.09957 0.08756;0.33667 0.22454 0.17196 0.12659 0.09928 0.08647;0.33518 0.22514 0.17187 0.12613 0.10014 0.08664;0.33524 0.22653 0.17256 0.1261 0.10082 0.08759;0.33556 0.22797 0.1733 0.12607 0.10155 0.0885;0.33589 0.22941 0.17405 0.12605 0.10227 0.08918;0.33622 0.23086 0.17484 0.12602 0.103 0.08985;0.33655 0.2323 0.1758 0.126 0.10373 0.09053;0.33688 0.23374 0.17676 0.12598 0.10446 0.0912;0.33721 0.23499 0.17772 0.12595 0.10519 0.09188;0.3381 0.23639 0.17924 0.12709 0.10648 0.09312;0.33905 0.23784 0.18082 0.12835 0.10783 0.09441;0.34 0.23929 0.18241 0.1296 0.10918 0.09571;0.34031 0.23991 0.18316 0.13037 0.1097 0.09618;0.34036 0.24011 0.18349 0.13088 0.1098 0.09608;0.3404 0.24031 0.18382 0.1314 0.10989 0.09597;0.3404 0.24047 0.1841 0.13182 0.10986 0.09581;0.34011 0.24033 0.1841 0.13158 0.10953 0.09535;0.33989 0.24027 0.18422 0.13136 0.10929 0.09498;0.34006 0.24021 0.18463 0.13113 0.10904 0.09461;0.34112 0.24015 0.18505 0.1309 0.1088 0.09423;0.34219 0.24057 0.18547 0.13069 0.10855 0.09385;0.34331 0.24158 0.18594 0.13059 0.10837 0.09322;0.34505 0.2432 0.18703 0.13086 0.10748 0.0932;0.348 0.24604 0.18933 0.13184 0.10774 0.09438;0.35095 0.24887 0.19163 0.13283 0.108 0.09557;0.35389 0.25171 0.19393 0.13381 0.10826 0.09676;0.35814 0.25442 0.19611 0.13455 0.1084 0.09783 ...(+755 chars)] % Datasheet derived Ohm  R0ThermalI=repmat([.0117, .0085, .009; .011, .0085, .009; .0114, .0087, .0092; .0107, .0082, .0088; .0107, .0083, .0091; .0113, .0085, .0089; .0116, .0085, .0089], 1, 1, 3) % Parameter not set Ohm  DischargeR0=[.0085, .0085, .0087, .0082, .0083, .0085, .0085] % Parameter not set Ohm  ChargeR0=[.0085, .0085, .0087, .0082, .0083, .0085, .0085] % Parameter not set Ohm  ChargeR0Thermal=[.0117, .0085, .009; .011, .0085, .009; .0114, .0087, .0092; .0107, .0082, .0088; .0107, .0083, .0091; .0113, .0085, .0089; .0116, .0085, .0089] % Parameter not set Ohm  DischargeR0Thermal=[.0117, .0085, .009; .011, .0085, .009; .0114, .0087, .0092; .0107, .0082, .0088; .0107, .0083, .0091; .0113, .0085, .0089; .0116, .0085, .0089] % Parameter not set Ohm  RCPairs=simscape.battery.enum.cells.RCPairs.noDynamics  R1=[.0029, .0024, .0026, .0016, .0023, .0018, .0017] % Parameter not set Ohm  Tau1=[36, 45, 105, 29, 77, 33, 39] % Parameter not set s  R2=[.0029, .0024, .0026, .0016, .0023, .0018, .0017] % Parameter not set Ohm  Tau2=[36, 45, 105, 29, 77, 33, 39] % Parameter not set s  R3=[.0029, .0024, .0026, .0016, .0023, .0018, .0017] % Parameter not set Ohm  Tau3=[36, 45, 105, 29, 77, 33, 39] % Parameter not set s  R1I=[.0109, .0029, .0013; .0069, .0024, .0012; .0047, .0026, .0013; .0034, .0016, .001; .0033, .0023, .0014; .0033, .0018, .0011; .0028, .0017, .0011] % Parameter not set Ohm  Tau1I=[20, 36, 39; 31, 45, 39; 109, 105, 61; 36, 29, 26; 59, 77, 67; 40, 33, 29; 25, 39, 33] % Parameter not set s  R2I=[.0109, .0029, .0013; .0069, .0024, .0012; .0047, .0026, .0013; .0034, .0016, .001; .0033, .0023, .0014; .0033, .0018, .0011; .0028, .0017, .0011] % Parameter not set Ohm  Tau2I=[20, 36, 39; 31, 45, 39; 109, 105, 61; 36, 29, 26; 59, 77, 67; 40, 33, 29; 25, 39, 33] % Parameter not set s  R3I=[.0109, .0029, .0013; .0069, .0024, .0012; .0047, .0026, .0013; .0034, .0016, .001; .0033, .0023, .0014; .0033, .0018, .0011; .0028, .0017, .0011] % Parameter not set Ohm  Tau3I=[20, 36, 39; 31, 45, 39; 109, 105, 61; 36, 29, 26; 59, 77, 67; 40, 33, 29; 25, 39, 33] % Parameter not set s  DischargeR1=[.0029, .0024, .0026, .0016, .0023, .0018, .0017] % Parameter not set Ohm  DischargeTau1=[36, 45, 105, 29, 77, 33, 39] % Parameter not set s  ChargeR1=[.0029, .0024, .0026, .0016, .0023, .0018, .0017] % Parameter not set Ohm  ChargeTau1=[36, 45, 105, 29, 77, 33, 39] % Parameter not set s  DischargeR2=[.0029, .0024, .0026, .0016, .0023, .0018, .0017] % Parameter not set Ohm  DischargeTau2=[36, 45, 105, 29, 77, 33, 39] % Parameter not set s  ChargeR2=[.0029, .0024, .0026, .0016, .0023, .0018, .0017] % Parameter not set Ohm  ChargeTau2=[36, 45, 105, 29, 77, 33, 39] % Parameter not set s  DischargeR3=[.0029, .0024, .0026, .0016, .0023, .0018, .0017] % Parameter not set Ohm  DischargeTau3=[36, 45, 105, 29, 77, 33, 39] % Parameter not set s  ChargeR3=[.0029, .0024, .0026, .0016, .0023, .0018, .0017] % Parameter not set Ohm  ChargeTau3=[36, 45, 105, 29, 77, 33, 39] % Parameter not set s  R1Thermal=[.0109, .0029, .0013; .0069, .0024, .0012; .0047, .0026, .0013; .0034, .0016, .001; .0033, .0023, .0014; .0033, .0018, .0011; .0028, .0017, .0011] % Parameter not set Ohm  Tau1Thermal=[20, 36, 39; 31, 45, 39; 109, 105, 61; 36, 29, 26; 59, 77, 67; 40, 33, 29; 25, 39, 33] % Parameter not set s  R2Thermal=[.0109, .0029, .0013; .0069, .0024, .0012; .0047, .0026, .0013; .0034, .0016, .001; .0033, .0023, .0014; .0033, .0018, .0011; .0028, .0017, .0011] % Parameter not set Ohm  Tau2Thermal=[20, 36, 39; 31, 45, 39; 109, 105, 61; 36, 29, 26; 59, 77, 67; 40, 33, 29; 25, 39, 33] % Parameter not set s  R3Thermal=[.0109, .0029, .0013; .0069, .0024, .0012; .0047, .0026, .0013; .0034, .0016, .001; .0033, .0023, .0014; .0033, .0018, .0011; .0028, .0017, .0011] % Parameter not set Ohm  Tau3Thermal=[20, 36, 39; 31, 45, 39; 109, 105, 61; 36, 29, 26; 59, 77, 67; 40, 33, 29; 25, 39, 33] % Parameter not set s  R1ThermalI=repmat([.0109, .0029, .0013; .0069, .0024, .0012; .0047, .0026, .0013; .0034, .0016, .001; .0033, .0023, .0014; .0033, .0018, .0011; .0028, .0017, .0011], 1, 1, 3) % Parameter not set Ohm  Tau1ThermalI=repmat([20, 36, 39; 31, 45, 39; 109, 105, 61; 36, 29, 26; 59, 77, 67; 40, 33, 29; 25, 39, 33], 1, 1, 3) % Parameter not set s  R2ThermalI=repmat([.0109, .0029, .0013; .0069, .0024, .0012; .0047, .0026, .0013; .0034, .0016, .001; .0033, .0023, .0014; .0033, .0018, .0011; .0028, .0017, .0011], 1, 1, 3) % Parameter not set Ohm  Tau2ThermalI=repmat([20, 36, 39; 31, 45, 39; 109, 105, 61; 36, 29, 26; 59, 77, 67; 40, 33, 29; 25, 39, 33], 1, 1, 3) % Parameter not set s  R3ThermalI=repmat([.0109, .0029, .0013; .0069, .0024, .0012; .0047, .0026, .0013; .0034, .0016, .001; .0033, .0023, .0014; .0033, .0018, .0011; .0028, .0017, .0011], 1, 1, 3) % Parameter not set Ohm  Tau3ThermalI=repmat([20, 36, 39; 31, 45, 39; 109, 105, 61; 36, 29, 26; 59, 77, 67; 40, 33, 29; 25, 39, 33], 1, 1, 3) % Parameter not set s  DischargeR1Thermal=[.0109, .0029, .0013; .0069, .0024, .0012; .0047, .0026, .0013; .0034, .0016, .001; .0033, .0023, .0014; .0033, .0018, .0011; .0028, .0017, .0011] % Parameter not set Ohm  DischargeTau1Thermal=[20, 36, 39; 31, 45, 39; 109, 105, 61; 36, 29, 26; 59, 77, 67; 40, 33, 29; 25, 39, 33] % Parameter not set s  ChargeR1Thermal=[.0109, .0029, .0013; .0069, .0024, .0012; .0047, .0026, .0013; .0034, .0016, .001; .0033, .0023, .0014; .0033, .0018, .0011; .0028, .0017, .0011] % Parameter not set Ohm  ChargeTau1Thermal=[20, 36, 39; 31, 45, 39; 109, 105, 61; 36, 29, 26; 59, 77, 67; 40, 33, 29; 25, 39, 33] % Parameter not set s  DischargeR2Thermal=[.0109, .0029, .0013; .0069, .0024, .0012; .0047, .0026, .0013; .0034, .0016, .001; .0033, .0023, .0014; .0033, .0018, .0011; .0028, .0017, .0011] % Parameter not set Ohm  DischargeTau2Thermal=[20, 36, 39; 31, 45, 39; 109, 105, 61; 36, 29, 26; 59, 77, 67; 40, 33, 29; 25, 39, 33] % Parameter not set s  ChargeR2Thermal=[.0109, .0029, .0013; .0069, .0024, .0012; .0047, .0026, .0013; .0034, .0016, .001; .0033, .0023, .0014; .0033, .0018, .0011; .0028, .0017, .0011] % Parameter not set Ohm  ChargeTau2Thermal=[20, 36, 39; 31, 45, 39; 109, 105, 61; 36, 29, 26; 59, 77, 67; 40, 33, 29; 25, 39, 33] % Parameter not set s  DischargeR3Thermal=[.0109, .0029, .0013; .0069, .0024, .0012; .0047, .0026, .0013; .0034, .0016, .001; .0033, .0023, .0014; .0033, .0018, .0011; .0028, .0017, .0011] % Parameter not set Ohm  DischargeTau3Thermal=[20, 36, 39; 31, 45, 39; 109, 105, 61; 36, 29, 26; 59, 77, 67; 40, 33, 29; 25, 39, 33] % Parameter not set s  ChargeR3Thermal=[.0109, .0029, .0013; .0069, .0024, .0012; .0047, .0026, .0013; .0034, .0016, .001; .0033, .0023, .0014; .0033, .0018, .0011; .0028, .0017, .0011] % Parameter not set Ohm  ChargeTau3Thermal=[20, 36, 39; 31, 45, 39; 109, 105, 61; 36, 29, 26; 59, 77, 67; 40, 33, 29; 25, 39, 33] % Parameter not set s  SelfDischargeResistor=simscape.battery.enum.cells.BatteryEnable.Disabled  SelfDischargeR=7e3 % Parameter not set Ohm  SelfDischargeRThermal=[8000, 7000, 6000] % Parameter not set Ohm  CyclingAgingMethod=simscape.battery.enum.cells.CyclingAgingMethod.tableN  CycleCalculationMethod=simscape.battery.enum.cells.CycleCalculationMethod.EquivalentCycles  NumDisCycles=100 % Parameter not set  OCVChange=0 % Parameter not set  R0Change=0 % Parameter not set  CapacityChange=0 % Parameter not set  SelfDischargeRChange=0 % Parameter not set  R1Change=0 % Parameter not set  R2Change=0 % Parameter not set  R3Change=0 % Parameter not set  NumDisCyclesBreakpoints=[0 7 13 19 25 31 37 43 49 55 61 67 73 79 85 91 97 103 109 115 121 127 133 139 145 151 157 163 169 175 181 187 193 199 205 211 217 223 229 235 241 247 253 259 265 271 277 283 289 295 301 307 313 319 325 331 337 343 349 355 361 367 373 379 385 391 397 403 409 415 421 427 433 439 445 451 457 463 469 475 481 487 493 499] % Datasheet derived  AgingTemperatureBreakpoints=[298.15, 323.15] % Parameter not set K  AgingCurrentBreakpoints=[-.1, -.5, -5] % Parameter not set A  OCVChangeVec=[0 -0.2056 -0.4112 -0.602 -0.7529 -0.9041 -1.0234 -1.116 -1.2087 -1.3013 -1.3939 -1.4865 -1.5404 -1.5936 -1.6468 -1.7 -1.7534 -1.807 -1.8607 -1.9143 -1.972 -2.0316 -2.0912 -2.1507 -2.2103 -2.2687 -2.3264 -2.3842 -2.442 -2.4996 -2.5474 -2.5914 -2.6354 -2.6795 -2.7235 -2.7676 -2.8116 -2.8556 -2.8997 -2.9437 -2.9899 -3.057 -3.1273 -3.1975 -3.2718 -3.347 -3.4222 -3.4977 -3.5744 -3.6428 -3.6945 -3.7461 -3.7966 -3.8466 -3.8965 -3.9465 -3.9964 -4.0461 -4.0951 -4.1498 -4.2072 -4.2646 -4.322 -4.3794 -4.4368 -4.4942 -4.5515 -4.61 -4.6685 -4.7269 -4.7854 -4.844 -4.9032 -4.9624 -5.0216 -5.0808 -5.1413 -5.2041 -5.2668 -5.3295 -5.3922 -5.455 -5.5177 -5.5804] % Datasheet derived  OCVChangeThermal=[0, 0; 0, 0; 0, 0; 0, 0] % Parameter not set  R0ChangeVec=[0 0 0 0 0 0 0 0 0 0 0 0 0 0 0 0 0 0 0 0 0 0 0 0 0 0 0 0 0 0 0 0 0 0 0 0 0 0 0 0 0 0 0 0 0 0 0 0 0 0 0 0 0 0 0 0 0 0 0 0 0 0 0 0 0 0 0 0 0 0 0 0 0 0 0 0 0 0 0 0 0 0 0 0] % Parameter assumed  R0ChangeThermal=[0, 0; 0, 0; 0, 0; 0, 0] % Parameter not set  R0ChangeThermalI=repmat(0, 4, 2, 3) % Parameter not set  R0CyclingChangeInitialTarget=0 % Parameter not set  CapacityChangeVec=[0 -0.367 -0.733 -1.1 -1.466 -1.834 -2.202 -2.571 -2.94 -3.309 -3.678 -4.047 -4.261 -4.473 -4.685 -4.897 -5.109 -5.32 -5.532 -5.744 -5.972 -6.21 -6.448 -6.686 -6.924 -7.162 -7.4 -7.638 -7.876 -8.114 -8.313 -8.496 -8.679 -8.862 -9.045 -9.228 -9.411 -9.593 -9.776 -9.959 -10.142 -10.405 -10.679 -10.954 -11.228 -11.503 -11.777 -12.052 -12.326 -12.571 -12.756 -12.941 -13.126 -13.311 -13.496 -13.681 -13.866 -14.051 -14.235 -14.442 -14.659 -14.875 -15.092 -15.308 -15.525 -15.741 -15.958 -16.175 -16.391 -16.607 -16.822 -17.038 -17.254 -17.47 -17.685 -17.901 -18.122 -18.35 -18.579 -18.807 -19.036 -19.265 -19.493 -19.722] % Datasheet derived  CapacityChangeThermal=[0, 0; 0, 0; 0, 0; 0, 0] % Parameter not set  CapacityChangeThermalI=repmat(0, 4, 2, 3) % Parameter not set  CapacityCyclingChangeInitialTarget=0 % Parameter not set  SelfDischargeRChangeVec=[0, 0, 0, 0] % Parameter not set  SelfDischargeRChangeThermal=[0, 0; 0, 0; 0, 0; 0, 0] % Parameter not set  SelfDischargeRChangeThermalI=repmat(0, 4, 2, 3) % Parameter not set  SelfDischargeRCyclingChangeInitialTarget=0 % Parameter not set  R1ChangeVec=[0, 0, 0, 0] % Parameter not set  R1ChangeThermal=[0, 0; 0, 0; 0, 0; 0, 0] % Parameter not set  R1ChangeThermalI=repmat(0, 4, 2, 3) % Parameter not set  R1CyclingChangeInitialTarget=0 % Parameter not set  R2ChangeVec=[0, 0, 0, 0] % Parameter not set  R2ChangeThermal=[0, 0; 0, 0; 0, 0; 0, 0] % Parameter not set  R2ChangeThermalI=repmat(0, 4, 2, 3) % Parameter not set  R2CyclingChangeInitialTarget=0 % Parameter not set  R3ChangeVec=[0, 0, 0, 0] % Parameter not set  R3ChangeThermal=[0, 0; 0, 0; 0, 0; 0, 0] % Parameter not set  R3ChangeThermalI=repmat(0, 4, 2, 3) % Parameter not set  R3CyclingChangeInitialTarget=0 % Parameter not set  CalendarAgeResistance=simscape.battery.enum.cells.BatteryEnable.Disabled  CalendarAgeCapacity=simscape.battery.enum.cells.BatteryEnable.Disabled  CalendarAgingMethod=simscape.battery.enum.cells.CalendarAgingMethod.equation  StorageVariable=simscape.battery.enum.cells.StorageVariable.OCV  OCVDuringStorage=0.9 % Parameter not set  SOCDuringStorage=0.6 % Parameter not set  StorageTimeIntervals=[0] % Parameter not set d  StorageTemperatures=[273] % Parameter not set K  ResistanceScalingOCV=2.2134e6 % Parameter not set  ResistanceScalingOCVOffset=1.632e6 % Parameter not set  ResistanceExponentialIncrease=0.515833569 % Parameter not set V  ResistanceTimeExponent=0.75 % Parameter not set  ResistanceAgeTemperatureBreakpoints=[273.15, 298.15, 323.15] % Parameter not set K  ResistanceAgeTimeBreakpoints=[0, 90, 180, 270] % Parameter not set d  PercentResistanceChange=[0, 0, 0] % Parameter not set  ResistanceTimeBreakpoints=100 % Parameter not set d  PercentResistanceChangeThermal=[0, 0, 0; 0, 0, 0; 0, 0, 0; 0, 0, 0] % Parameter not set  CapacityScalingOCV=1.5097e07 % Parameter not set  CapacityScalingOCVOffset=8.3625e06 % Parameter not set  CapacityExponentialIncrease=0.6011 % Parameter not set V  CapacityTimeExponent=0.75 % Parameter not set  CapacityAgeTemperatureBreakpoints=[273.15, 298.15, 323.15] % Parameter not set K  CapacityAgeTimeBreakpoints=[0, 90, 180, 270] % Parameter not set d  PercentCapacityChange=[0, 0, 0] % Parameter not set  CapacityTimeBreakpoints=100 % Parameter not set d  PercentCapacityChangeThermal=[0, 0, 0; 0, 0, 0; 0, 0, 0; 0, 0, 0] % Parameter not set  SimulationTemperature=298.15 % Parameter not set K  BatteryThermalMass=20.7 % Parameter assumed J/K  NumThermalModels=6 % Parameter not set  ThermalConductivityZ=18 % Parameter not set W/(K*m)  CrossSectionalAreaXY=0.000286 m^2  Height=0.036 m  ReversibleHeatModel=simscape.battery.enum.cells.ReversibleHeatModel.Disabled  EntropicCoefficient=[0, 0, 0, 0, 0, 0, 0] % Parameter not set mV/K  CurrentDirectionality=simscape.battery.enum.cells.BatteryEnable.Disabled  stateOfCharge_specify=off  stateOfCharge_priority=High  stateOfCharge=1  stateOfCharge_nominal_specify=off  stateOfCharge_nominal_value=1  stateOfCharge_nominal_unit=1  batteryVoltage_specify=off  batteryVoltage_priority=Low  batteryVoltage=3 V  batteryVoltage_nominal_specify=off  batteryVoltage_nominal_value=1  batteryVoltage_nominal_unit=V  batteryCurrent_specify=off  batteryCurrent_priority=None  batteryCurrent=0 A  batteryCurrent_nominal_specify=off  batteryCurrent_nominal_value=1  batteryCurrent_nominal_unit=A  numCycles_specify=off  numCycles_priority=High  numCycles=0  numCycles_nominal_specify=off  numCycles_nominal_value=1  numCycles_nominal_unit=1  batteryTemperature_specify=off  batteryTemperature_priority=High  batteryTemperature=298.15 K  batteryTemperature_nominal_specify=off  batteryTemperature_nominal_value=1  batteryTemperature_nominal_unit=K  hysteresisState_specify=off  hysteresisState_priority=High  hysteresisState=0  hysteresisState_nominal_specify=off  hysteresisState_nominal_value=1  hysteresisState_nominal_unit=1  isExothermFaulted_specify=off  isExothermFaulted_priority=None  isExothermFaulted=0  isExothermFaulted_nominal_specify=off  isExothermFaulted_nominal_value=1  isExothermFaulted_nominal_unit=1  reactionHeatRate_specify=off  reactionHeatRate_priority=None  reactionHeatRate=0 W  reactionHeatRate_nominal_specify=off  reactionHeatRate_nominal_value=1  reactionHeatRate_nominal_unit=W  reactionExtent_specify=off  reactionExtent_priority=None  reactionExtent=0  reactionExtent_nominal_specify=off  reactionExtent_nominal_value=1  reactionExtent_nominal_unit=1
      settings: AttributesFormatString=Panasonic:NCA843436  InternalSimscapePortConfiguration="{\"Bottom\":[{\"id\":\"n\",\"label\":\"-\",\"type\":\"foundation.electrical.electrical\"},{\"id\":\"H\",\"label\":\"H\",\"type\":\"foundation.thermal.thermal\"}],\"Left\":[],\"Right\":[],\"Top\":[{\"id\":\"p\",\"label\":\"+\",\"type\":\"foundation.electrical.electrical\"}]}"
  Battery Equivalent Circuit8 : batt_lib/Cells/Battery Equivalent Circuit  PartSpecification="{\"CollectionId\":\"SimscapeBattery\",\"CollectionVersion\":\"1.0.0\",\"DatasetId\":\"Panasonic|NCA843436|simscape.battery.batteryEquivalentCircuit\",\"DisplayName\":\"Panasonic:NCA843436\"}"  BatteryCapacity=1.354 % Datasheet derived hr*A  ThermalModel=simscape.battery.enum.cells.BatteryThermalModel.LumpedThermalMass  ExtrapolationMethod=simscape.enum.extrapolation.linear  SOCBreakpoints=[0 0.01 0.02 0.03 0.04 0.05 0.06 0.07 0.08 0.09 0.1 0.11 0.12 0.13 0.14 0.15 0.16 0.17 0.18 0.19 0.2 0.21 0.22 0.23 0.24 0.25 0.26 0.27 0.28 0.29 0.3 0.31 0.32 0.33 0.34 0.35 0.36 0.37 0.38 0.39 0.4 0.41 0.42 0.43 0.44 0.45 0.46 0.47 0.48 0.49 0.5 0.51 0.52 0.53 0.54 0.55 0.56 0.57 0.58 0.59 0.6 0.61 0.62 0.63 0.64 0.65 0.66 0.67 0.68 0.69 0.7 0.71 0.72 0.73 0.74 0.75 0.76 0.77 0.78 0.79 0.8 0.81 0.82 0.83 0.84 0.85 0.86 0.87 0.88 0.89 0.9 0.91 0.92 0.93 0.94 0.95 0.96 0.97 0.98 0.99 1] % Datasheet derived  TemperatureBreakpoints=[-10 0 10 25 45 60] % Datasheet derived degC  OpenCircuitVoltage=[2.817 2.94537 3.0182 3.08984 3.15197 3.18868 3.22389 3.25188 3.27953 3.3028 3.32214 3.34136 3.36247 3.37682 3.38851 3.4018 3.4147 3.42636 3.43803 3.44822 3.45549 3.46277 3.47005 3.47732 3.4846 3.49328 3.49997 3.50631 3.51243 3.51855 3.52468 3.5308 3.53692 3.54304 3.54917 3.55568 3.56257 3.56948 3.57636 3.58289 3.58942 3.59595 3.60248 3.60901 3.61554 3.62207 3.62861 3.63511 3.64233 3.65 3.65825 3.6665 3.67476 3.68301 3.69126 3.69952 3.70777 3.71583 3.72334 3.73246 3.74258 3.75276 3.76295 3.77313 3.78331 3.7935 3.80368 3.81459 3.82556 3.83654 3.84646 3.85584 3.86522 3.87454 3.8835 3.89255 3.9016 3.91065 3.91971 3.92884 3.93875 3.95021 3.96167 3.97312 3.98443 3.99549 4.00655 4.01783 4.0295 4.04093 4.05161 4.06166 4.07171 4.08185 4.09229 4.10286 4.11335 4.12383 4.13431 4.1515 4.17492] % Datasheet derived V  OpenCircuitVoltageThermal=[2.817 2.817 2.817 2.817 2.817 2.817;2.94537 2.94537 2.94537 2.94537 2.94537 2.94537;3.0182 3.0182 3.0182 3.0182 3.0182 3.0182;3.08984 3.08984 3.08984 3.08984 3.08984 3.08984;3.15197 3.15197 3.15197 3.15197 3.15197 3.15197;3.18868 3.18868 3.18868 3.18868 3.18868 3.18868;3.22389 3.22389 3.22389 3.22389 3.22389 3.22389;3.25188 3.25188 3.25188 3.25188 3.25188 3.25188;3.27953 3.27953 3.27953 3.27953 3.27953 3.27953;3.3028 3.3028 3.3028 3.3028 3.3028 3.3028;3.32214 3.32214 3.32214 3.32214 3.32214 3.32214;3.34136 3.34136 3.34136 3.34136 3.34136 3.34136;3.36247 3.36247 3.36247 3.36247 3.36247 3.36247;3.37682 3.37682 3.37682 3.37682 3.37682 3.37682;3.38851 3.38851 3.38851 3.38851 3.38851 3.38851;3.4018 3.4018 3.4018 3.4018 3.4018 3.4018;3.4147 3.4147 3.4147 3.4147 3.4147 3.4147;3.42636 3.42636 3.42636 3.42636 3.42636 3.42636;3.43803 3.43803 3.43803 3.43803 3.43803 3.43803;3.44822 3.44822 3.44822 3.44822 3.44822 3.44822;3.45549 3.45549 3.45549 3.45549 3.45549 3.45549;3.46277 3.46277 3.46277 3.46277 3.46277 3.46277;3.47005 3.47005 3.47005 3.47005 3.47005 3.47005;3.47732 3.47732 3.47732 3.47732 3.47732 3.47732;3.4846 3.4846 3.4846 3.4846 3.4846 3.4846;3.49328 3.49328 3.49328 3.49328 3.49328 3.49328;3.49997 3.49997 3.49997 3.49997 3.49997 3.49997;3.50631 3.50631 3.50631 3.50631 3.50631 3.50631;3.51243 3.51243 3.51243 3.51243 3.51243 3.51243;3.51855 3.51855 3.51855 3.51855 3.51855 3.51855;3.52468 3.52468 3.52468 3.52468 3.52468 3.52468;3.5308 3.5308 3.5308 3.5308 3.5308 3.5308;3.53692 3.53692 3.53692 3.53692 3.53692 3.53692;3.54304 3.54304 3.54304 3.54304 3.54304 3.54304;3.54917 3.54917 3.54917 3.54917 3.54917 3.54917;3.55568 3.55568 3.55568 3.55568 3.55568 3.55568;3.56257 3.56257 3.56257 3.56257 3.56257 3.56257;3.56948 3.56948 3.56948 3.56948 3.56948 3.56948;3.57636 3.57636 3.57636 3.57636 3.57636 3.57636;3.58289 3.58289 3.58289 3.58289 3.58289 3.58289;3.58942 3.58942 3.58942 3.58942 3.58942 3.58942;3.59595 3.59595 3.59595 3.59595 3.59595 3.59595;3.60248 3.60248 3.60248 3.60248 3.60248 3.60248;3.60901 3.60901 3.60901 3.60901 3.60901 3.60901;3.61554 3.61554 3.61554 3.61554 3.61554 3.61554;3.62207 3.62207 3.62207 3.62207 3.62207 3.62207;3.62861 3.62861 3.62861 3.62861 3.62861 3.62861;3.63511 3.63511 3.63511 3.63511 3.63511 3.63511;3.64233 3.64233 3.64233 3.64233 3.64233 3.64233;3.65 3.65 3.65 3.65 3.65 3.65;3.65825 3.65825 3.65825 3.65825 3.65825 3.65825;3.6665 3.6665 3.6665 3.6665 3.6665 3.6665;3.67476 3.67476 3.67476 3.67476 3.67476 3.67476;3.68301 3.68301 3.68301 3.68301 3.68301 3.68301;3.69126 3.69126 3.69126 3.69126 3.69126 3.69126;3.69952 3.69952 3.69952 3.69952 3.69952 3.69952;3.70777 3.70777 3.70777 3.70777 3.70777 3.70777;3.71583 3.71583 3.71583 3.71583 3.71583 3.71583;3.72334 3.72334 3.72334 3.72334 3.72334 3.72334;3.73246 3.73246 3.73246 3.73246 3.73246 3.73246;3.74258 3.74258 3.74258 3.74258 3.74258 3.74258;3.75276 3.75276 3.75276 3.75276 3.75276 3.75276;3.76295 3.76295 3.76295 3.76295 3.76295 3.76295;3.77313 3.77313 3.77313 3.77313 3.77313 3.77313;3.78331 3.78331 3.78331 3.78331 3.78331 3.78331;3.7935 3.7935 3.7935 3.7935 3.7935 3.7935;3.80368 3.80368 3.80368 3.80368 3.80368 3.80368;3.81459 3.81459 3.81459 3.81459 3.81459 3.81459;3.82556 3.82556 3.82556 3.82556 3.82556 3.82556;3.83654 3.83654 3.83654 3.83654 3.83654 3.83654;3.84646 3.84646 3.84646 3.84646 3.84646 3.84646;3.85584 3.85584 3.85584 3.85584 3.85584 3.85584;3.86522 3.86522 3.86522 3.86522 3.86522 3.86522;3.87454 3.87454 3.87454 3.87454 3.87454 3.87454;3.8835 3.8835 3.8835 3.8835 3.8835 3.8835;3.89255 3.89255 3.89255 3.89255 3.89255 3.89255;3.9016 3.9016 3.9016 3.9016 3.9016 3.9016;3.91065 3.91065 3.91065 3.91065 3.91065 3.91065;3.91971 3.91971 3.91971 3.91971 3.91971 3.91971;3.92884 3.92884 3.92884 3.92884 3.92884 3.92884;3.93875 3.93875 3.93875 3.93875 3.93875 3.93875;3.95021 3.95021 3.95021 3.95021 3.95021 3.95021;3.96167 3.96167 3.96167 3.96167 3.96167 3.96167;3.97312 3.97312 3.97312 3.97312 3.97312 3.97312;3.98443 3.98443 3.98443 3.98443 3.98443 3.98443;3.99549 ...(+748 chars)] % Datasheet derived V  VoltageRange=[2.25 Inf] % Datasheet derived V  HysteresisModel=simscape.battery.enum.cells.HysteresisModel.none  MaximumHysteresisVoltage=[0, 0, 0, 0, 0, 0, 0] % Parameter not set V  InstantaneousHysteresisVoltage=[0, 0, 0, 0, 0, 0, 0] % Parameter not set V  HysteresisRate=0.1 % Parameter not set  MaximumHysteresisVoltageThermal=[0, 0, 0; 0, 0, 0; 0, 0, 0; 0, 0, 0; 0, 0, 0; 0, 0, 0; 0, 0, 0] % Parameter not set V  InstantaneousHysteresisVoltageThermal=[0, 0, 0; 0, 0, 0; 0, 0, 0; 0, 0, 0; 0, 0, 0; 0, 0, 0; 0, 0, 0] % Parameter not set V  HysteresisRateThermal=0.1 % Parameter not set  ResistanceSOCBreakpoints=[0 0.01 0.02 0.03 0.04 0.05 0.06 0.07 0.08 0.09 0.1 0.11 0.12 0.13 0.14 0.15 0.16 0.17 0.18 0.19 0.2 0.21 0.22 0.23 0.24 0.25 0.26 0.27 0.28 0.29 0.3 0.31 0.32 0.33 0.34 0.35 0.36 0.37 0.38 0.39 0.4 0.41 0.42 0.43 0.44 0.45 0.46 0.47 0.48 0.49 0.5 0.51 0.52 0.53 0.54 0.55 0.56 0.57 0.58 0.59 0.6 0.61 0.62 0.63 0.64 0.65 0.66 0.67 0.68 0.69 0.7 0.71 0.72 0.73 0.74 0.75 0.76 0.77 0.78 0.79 0.8 0.81 0.82 0.83 0.84 0.85 0.86 0.87 0.88 0.89 0.9 0.91 0.92 0.93 0.94 0.95 0.96 0.97 0.98 0.99 1] % Datasheet derived  ResistanceTemperatureBreakpoints=[-10 0 10 25 45 60] % Datasheet derived degC  ResistanceCurrentBreakpoints=[-1, 0, 1] % Parameter not set A  CurrentDependence=simscape.battery.enum.cells.CurrentDependence.Disabled  R0=[0.31638 0.3243 0.30647 0.2881 0.26534 0.23483 0.21466 0.1963 0.19065 0.18321 0.17517 0.17035 0.1686 0.16602 0.16263 0.16182 0.16098 0.16003 0.15908 0.15746 0.15485 0.15224 0.14963 0.14702 0.14441 0.14408 0.14309 0.14204 0.14098 0.13992 0.13886 0.13779 0.13673 0.13567 0.13461 0.13373 0.13328 0.13287 0.13246 0.13202 0.13158 0.13114 0.1307 0.13026 0.12982 0.12938 0.12894 0.12846 0.12829 0.12823 0.12821 0.1282 0.12818 0.12817 0.12815 0.12814 0.12812 0.12779 0.12659 0.12613 0.1261 0.12607 0.12605 0.12602 0.126 0.12598 0.12595 0.12709 0.12835 0.1296 0.13037 0.13088 0.1314 0.13182 0.13158 0.13136 0.13113 0.1309 0.13069 0.13059 0.13086 0.13184 0.13283 0.13381 0.13455 0.1349 0.13525 0.13561 0.13601 0.1363 0.13601 0.1347 0.13339 0.13211 0.13099 0.12903 0.12626 0.1235 0.12073 0.11181 0.10295] % Datasheet derived Ohm  R0I=[.0117, .0085, .009; .011, .0085, .009; .0114, .0087, .0092; .0107, .0082, .0088; .0107, .0083, .0091; .0113, .0085, .0089; .0116, .0085, .0089] % Parameter not set Ohm  R0Thermal=[1.5461 1.75516 2.11759 0.31638 0.46651 0.23498;1.5461 1.99954 2.27305 0.3243 0.34615 0.09965;1.5461 1.92281 2.1374 0.30647 0.20343 0.05211;1.5461 1.84609 2.00176 0.2881 0.15069 0.02648;1.5461 1.76937 1.86611 0.26534 0.12351 0.03545;1.5461 1.69264 1.73046 0.23483 0.10579 0.0319;1.5461 1.61592 1.59482 0.21466 0.09923 0.03983;1.5461 1.5392 1.45917 0.1963 0.0958 0.05105;1.5461 1.46247 1.32352 0.19065 0.10282 0.06344;1.5461 1.38575 1.18787 0.18321 0.10641 0.07241;1.5461 1.30902 1.05223 0.17517 0.10811 0.07828;1.5461 1.2323 0.91658 0.17035 0.11082 0.08499;1.5461 1.15558 0.78093 0.1686 0.11501 0.09321;1.50339 1.07885 0.64529 0.16602 0.11389 0.09611;1.46067 1.00213 0.52896 0.16263 0.11281 0.09693;1.41796 0.92541 0.45732 0.16182 0.1148 0.09886;1.37525 0.84868 0.40356 0.16098 0.11649 0.10041;1.33254 0.77196 0.35633 0.16003 0.1172 0.10099;1.28982 0.69523 0.32513 0.15908 0.11792 0.10158;1.24711 0.61749 0.29756 0.15746 0.11748 0.101;1.2044 0.5576 0.27681 0.15485 0.11475 0.09814;1.16169 0.50708 0.25953 0.15224 0.11202 0.09528;1.11897 0.46758 0.24304 0.14963 0.11054 0.09242;1.07626 0.43256 0.23145 0.14702 0.10939 0.09016;1.03355 0.40213 0.21986 0.14441 0.10825 0.08946;0.99084 0.37836 0.21479 0.14408 0.10821 0.08986;0.94812 0.35585 0.21092 0.14309 0.1066 0.08869;0.90541 0.33652 0.20677 0.14204 0.10481 0.08725;0.8627 0.32218 0.20275 0.14098 0.10391 0.08564;0.81999 0.30785 0.19912 0.13992 0.10301 0.08404;0.77727 0.29756 0.19549 0.13886 0.1021 0.08274;0.73457 0.28818 0.19186 0.13779 0.10125 0.08295;0.69186 0.2788 0.1889 0.13673 0.10088 0.08317;0.65043 0.27154 0.18649 0.13567 0.10051 0.08339;0.60913 0.26481 0.18408 0.13461 0.10013 0.0836;0.57538 0.25838 0.18198 0.13373 0.10007 0.08413;0.5481 0.25225 0.18022 0.13328 0.10029 0.08494;0.52084 0.24869 0.17996 0.13287 0.10054 0.08577;0.49467 0.24569 0.17968 0.13246 0.10076 0.08658;0.47265 0.24242 0.17912 0.13202 0.10071 0.08711;0.45063 0.23914 0.17856 0.13158 0.10065 0.08708;0.43278 0.23587 0.17801 0.13114 0.10056 0.08706;0.42113 0.23372 0.17745 0.1307 0.09993 0.08703;0.40948 0.23194 0.17689 0.13026 0.09931 0.087;0.39802 0.23016 0.17625 0.12982 0.09869 0.08698;0.3895 0.22838 0.17554 0.12938 0.09807 0.08695;0.38098 0.2266 0.17484 0.12894 0.09745 0.08692;0.37243 0.2248 0.17411 0.12846 0.09681 0.08688;0.36446 0.22399 0.17395 0.12829 0.09673 0.08739;0.35683 0.2238 0.17413 0.12823 0.097 0.08826;0.35467 0.22407 0.17478 0.12821 0.09771 0.08958;0.35251 0.22433 0.17543 0.1282 0.098 0.09079;0.35035 0.2246 0.17607 0.12818 0.09829 0.09028;0.34819 0.22487 0.17654 0.12817 0.09857 0.08977;0.34604 0.22513 0.17577 0.12815 0.09886 0.08925;0.34388 0.2254 0.175 0.12814 0.09915 0.08874;0.34172 0.22541 0.17423 0.12812 0.09944 0.08823;0.3394 0.22519 0.17331 0.12779 0.09957 0.08756;0.33667 0.22454 0.17196 0.12659 0.09928 0.08647;0.33518 0.22514 0.17187 0.12613 0.10014 0.08664;0.33524 0.22653 0.17256 0.1261 0.10082 0.08759;0.33556 0.22797 0.1733 0.12607 0.10155 0.0885;0.33589 0.22941 0.17405 0.12605 0.10227 0.08918;0.33622 0.23086 0.17484 0.12602 0.103 0.08985;0.33655 0.2323 0.1758 0.126 0.10373 0.09053;0.33688 0.23374 0.17676 0.12598 0.10446 0.0912;0.33721 0.23499 0.17772 0.12595 0.10519 0.09188;0.3381 0.23639 0.17924 0.12709 0.10648 0.09312;0.33905 0.23784 0.18082 0.12835 0.10783 0.09441;0.34 0.23929 0.18241 0.1296 0.10918 0.09571;0.34031 0.23991 0.18316 0.13037 0.1097 0.09618;0.34036 0.24011 0.18349 0.13088 0.1098 0.09608;0.3404 0.24031 0.18382 0.1314 0.10989 0.09597;0.3404 0.24047 0.1841 0.13182 0.10986 0.09581;0.34011 0.24033 0.1841 0.13158 0.10953 0.09535;0.33989 0.24027 0.18422 0.13136 0.10929 0.09498;0.34006 0.24021 0.18463 0.13113 0.10904 0.09461;0.34112 0.24015 0.18505 0.1309 0.1088 0.09423;0.34219 0.24057 0.18547 0.13069 0.10855 0.09385;0.34331 0.24158 0.18594 0.13059 0.10837 0.09322;0.34505 0.2432 0.18703 0.13086 0.10748 0.0932;0.348 0.24604 0.18933 0.13184 0.10774 0.09438;0.35095 0.24887 0.19163 0.13283 0.108 0.09557;0.35389 0.25171 0.19393 0.13381 0.10826 0.09676;0.35814 0.25442 0.19611 0.13455 0.1084 0.09783 ...(+755 chars)] % Datasheet derived Ohm  R0ThermalI=repmat([.0117, .0085, .009; .011, .0085, .009; .0114, .0087, .0092; .0107, .0082, .0088; .0107, .0083, .0091; .0113, .0085, .0089; .0116, .0085, .0089], 1, 1, 3) % Parameter not set Ohm  DischargeR0=[.0085, .0085, .0087, .0082, .0083, .0085, .0085] % Parameter not set Ohm  ChargeR0=[.0085, .0085, .0087, .0082, .0083, .0085, .0085] % Parameter not set Ohm  ChargeR0Thermal=[.0117, .0085, .009; .011, .0085, .009; .0114, .0087, .0092; .0107, .0082, .0088; .0107, .0083, .0091; .0113, .0085, .0089; .0116, .0085, .0089] % Parameter not set Ohm  DischargeR0Thermal=[.0117, .0085, .009; .011, .0085, .009; .0114, .0087, .0092; .0107, .0082, .0088; .0107, .0083, .0091; .0113, .0085, .0089; .0116, .0085, .0089] % Parameter not set Ohm  RCPairs=simscape.battery.enum.cells.RCPairs.noDynamics  R1=[.0029, .0024, .0026, .0016, .0023, .0018, .0017] % Parameter not set Ohm  Tau1=[36, 45, 105, 29, 77, 33, 39] % Parameter not set s  R2=[.0029, .0024, .0026, .0016, .0023, .0018, .0017] % Parameter not set Ohm  Tau2=[36, 45, 105, 29, 77, 33, 39] % Parameter not set s  R3=[.0029, .0024, .0026, .0016, .0023, .0018, .0017] % Parameter not set Ohm  Tau3=[36, 45, 105, 29, 77, 33, 39] % Parameter not set s  R1I=[.0109, .0029, .0013; .0069, .0024, .0012; .0047, .0026, .0013; .0034, .0016, .001; .0033, .0023, .0014; .0033, .0018, .0011; .0028, .0017, .0011] % Parameter not set Ohm  Tau1I=[20, 36, 39; 31, 45, 39; 109, 105, 61; 36, 29, 26; 59, 77, 67; 40, 33, 29; 25, 39, 33] % Parameter not set s  R2I=[.0109, .0029, .0013; .0069, .0024, .0012; .0047, .0026, .0013; .0034, .0016, .001; .0033, .0023, .0014; .0033, .0018, .0011; .0028, .0017, .0011] % Parameter not set Ohm  Tau2I=[20, 36, 39; 31, 45, 39; 109, 105, 61; 36, 29, 26; 59, 77, 67; 40, 33, 29; 25, 39, 33] % Parameter not set s  R3I=[.0109, .0029, .0013; .0069, .0024, .0012; .0047, .0026, .0013; .0034, .0016, .001; .0033, .0023, .0014; .0033, .0018, .0011; .0028, .0017, .0011] % Parameter not set Ohm  Tau3I=[20, 36, 39; 31, 45, 39; 109, 105, 61; 36, 29, 26; 59, 77, 67; 40, 33, 29; 25, 39, 33] % Parameter not set s  DischargeR1=[.0029, .0024, .0026, .0016, .0023, .0018, .0017] % Parameter not set Ohm  DischargeTau1=[36, 45, 105, 29, 77, 33, 39] % Parameter not set s  ChargeR1=[.0029, .0024, .0026, .0016, .0023, .0018, .0017] % Parameter not set Ohm  ChargeTau1=[36, 45, 105, 29, 77, 33, 39] % Parameter not set s  DischargeR2=[.0029, .0024, .0026, .0016, .0023, .0018, .0017] % Parameter not set Ohm  DischargeTau2=[36, 45, 105, 29, 77, 33, 39] % Parameter not set s  ChargeR2=[.0029, .0024, .0026, .0016, .0023, .0018, .0017] % Parameter not set Ohm  ChargeTau2=[36, 45, 105, 29, 77, 33, 39] % Parameter not set s  DischargeR3=[.0029, .0024, .0026, .0016, .0023, .0018, .0017] % Parameter not set Ohm  DischargeTau3=[36, 45, 105, 29, 77, 33, 39] % Parameter not set s  ChargeR3=[.0029, .0024, .0026, .0016, .0023, .0018, .0017] % Parameter not set Ohm  ChargeTau3=[36, 45, 105, 29, 77, 33, 39] % Parameter not set s  R1Thermal=[.0109, .0029, .0013; .0069, .0024, .0012; .0047, .0026, .0013; .0034, .0016, .001; .0033, .0023, .0014; .0033, .0018, .0011; .0028, .0017, .0011] % Parameter not set Ohm  Tau1Thermal=[20, 36, 39; 31, 45, 39; 109, 105, 61; 36, 29, 26; 59, 77, 67; 40, 33, 29; 25, 39, 33] % Parameter not set s  R2Thermal=[.0109, .0029, .0013; .0069, .0024, .0012; .0047, .0026, .0013; .0034, .0016, .001; .0033, .0023, .0014; .0033, .0018, .0011; .0028, .0017, .0011] % Parameter not set Ohm  Tau2Thermal=[20, 36, 39; 31, 45, 39; 109, 105, 61; 36, 29, 26; 59, 77, 67; 40, 33, 29; 25, 39, 33] % Parameter not set s  R3Thermal=[.0109, .0029, .0013; .0069, .0024, .0012; .0047, .0026, .0013; .0034, .0016, .001; .0033, .0023, .0014; .0033, .0018, .0011; .0028, .0017, .0011] % Parameter not set Ohm  Tau3Thermal=[20, 36, 39; 31, 45, 39; 109, 105, 61; 36, 29, 26; 59, 77, 67; 40, 33, 29; 25, 39, 33] % Parameter not set s  R1ThermalI=repmat([.0109, .0029, .0013; .0069, .0024, .0012; .0047, .0026, .0013; .0034, .0016, .001; .0033, .0023, .0014; .0033, .0018, .0011; .0028, .0017, .0011], 1, 1, 3) % Parameter not set Ohm  Tau1ThermalI=repmat([20, 36, 39; 31, 45, 39; 109, 105, 61; 36, 29, 26; 59, 77, 67; 40, 33, 29; 25, 39, 33], 1, 1, 3) % Parameter not set s  R2ThermalI=repmat([.0109, .0029, .0013; .0069, .0024, .0012; .0047, .0026, .0013; .0034, .0016, .001; .0033, .0023, .0014; .0033, .0018, .0011; .0028, .0017, .0011], 1, 1, 3) % Parameter not set Ohm  Tau2ThermalI=repmat([20, 36, 39; 31, 45, 39; 109, 105, 61; 36, 29, 26; 59, 77, 67; 40, 33, 29; 25, 39, 33], 1, 1, 3) % Parameter not set s  R3ThermalI=repmat([.0109, .0029, .0013; .0069, .0024, .0012; .0047, .0026, .0013; .0034, .0016, .001; .0033, .0023, .0014; .0033, .0018, .0011; .0028, .0017, .0011], 1, 1, 3) % Parameter not set Ohm  Tau3ThermalI=repmat([20, 36, 39; 31, 45, 39; 109, 105, 61; 36, 29, 26; 59, 77, 67; 40, 33, 29; 25, 39, 33], 1, 1, 3) % Parameter not set s  DischargeR1Thermal=[.0109, .0029, .0013; .0069, .0024, .0012; .0047, .0026, .0013; .0034, .0016, .001; .0033, .0023, .0014; .0033, .0018, .0011; .0028, .0017, .0011] % Parameter not set Ohm  DischargeTau1Thermal=[20, 36, 39; 31, 45, 39; 109, 105, 61; 36, 29, 26; 59, 77, 67; 40, 33, 29; 25, 39, 33] % Parameter not set s  ChargeR1Thermal=[.0109, .0029, .0013; .0069, .0024, .0012; .0047, .0026, .0013; .0034, .0016, .001; .0033, .0023, .0014; .0033, .0018, .0011; .0028, .0017, .0011] % Parameter not set Ohm  ChargeTau1Thermal=[20, 36, 39; 31, 45, 39; 109, 105, 61; 36, 29, 26; 59, 77, 67; 40, 33, 29; 25, 39, 33] % Parameter not set s  DischargeR2Thermal=[.0109, .0029, .0013; .0069, .0024, .0012; .0047, .0026, .0013; .0034, .0016, .001; .0033, .0023, .0014; .0033, .0018, .0011; .0028, .0017, .0011] % Parameter not set Ohm  DischargeTau2Thermal=[20, 36, 39; 31, 45, 39; 109, 105, 61; 36, 29, 26; 59, 77, 67; 40, 33, 29; 25, 39, 33] % Parameter not set s  ChargeR2Thermal=[.0109, .0029, .0013; .0069, .0024, .0012; .0047, .0026, .0013; .0034, .0016, .001; .0033, .0023, .0014; .0033, .0018, .0011; .0028, .0017, .0011] % Parameter not set Ohm  ChargeTau2Thermal=[20, 36, 39; 31, 45, 39; 109, 105, 61; 36, 29, 26; 59, 77, 67; 40, 33, 29; 25, 39, 33] % Parameter not set s  DischargeR3Thermal=[.0109, .0029, .0013; .0069, .0024, .0012; .0047, .0026, .0013; .0034, .0016, .001; .0033, .0023, .0014; .0033, .0018, .0011; .0028, .0017, .0011] % Parameter not set Ohm  DischargeTau3Thermal=[20, 36, 39; 31, 45, 39; 109, 105, 61; 36, 29, 26; 59, 77, 67; 40, 33, 29; 25, 39, 33] % Parameter not set s  ChargeR3Thermal=[.0109, .0029, .0013; .0069, .0024, .0012; .0047, .0026, .0013; .0034, .0016, .001; .0033, .0023, .0014; .0033, .0018, .0011; .0028, .0017, .0011] % Parameter not set Ohm  ChargeTau3Thermal=[20, 36, 39; 31, 45, 39; 109, 105, 61; 36, 29, 26; 59, 77, 67; 40, 33, 29; 25, 39, 33] % Parameter not set s  SelfDischargeResistor=simscape.battery.enum.cells.BatteryEnable.Disabled  SelfDischargeR=7e3 % Parameter not set Ohm  SelfDischargeRThermal=[8000, 7000, 6000] % Parameter not set Ohm  CyclingAgingMethod=simscape.battery.enum.cells.CyclingAgingMethod.tableN  CycleCalculationMethod=simscape.battery.enum.cells.CycleCalculationMethod.EquivalentCycles  NumDisCycles=100 % Parameter not set  OCVChange=0 % Parameter not set  R0Change=0 % Parameter not set  CapacityChange=0 % Parameter not set  SelfDischargeRChange=0 % Parameter not set  R1Change=0 % Parameter not set  R2Change=0 % Parameter not set  R3Change=0 % Parameter not set  NumDisCyclesBreakpoints=[0 7 13 19 25 31 37 43 49 55 61 67 73 79 85 91 97 103 109 115 121 127 133 139 145 151 157 163 169 175 181 187 193 199 205 211 217 223 229 235 241 247 253 259 265 271 277 283 289 295 301 307 313 319 325 331 337 343 349 355 361 367 373 379 385 391 397 403 409 415 421 427 433 439 445 451 457 463 469 475 481 487 493 499] % Datasheet derived  AgingTemperatureBreakpoints=[298.15, 323.15] % Parameter not set K  AgingCurrentBreakpoints=[-.1, -.5, -5] % Parameter not set A  OCVChangeVec=[0 -0.2056 -0.4112 -0.602 -0.7529 -0.9041 -1.0234 -1.116 -1.2087 -1.3013 -1.3939 -1.4865 -1.5404 -1.5936 -1.6468 -1.7 -1.7534 -1.807 -1.8607 -1.9143 -1.972 -2.0316 -2.0912 -2.1507 -2.2103 -2.2687 -2.3264 -2.3842 -2.442 -2.4996 -2.5474 -2.5914 -2.6354 -2.6795 -2.7235 -2.7676 -2.8116 -2.8556 -2.8997 -2.9437 -2.9899 -3.057 -3.1273 -3.1975 -3.2718 -3.347 -3.4222 -3.4977 -3.5744 -3.6428 -3.6945 -3.7461 -3.7966 -3.8466 -3.8965 -3.9465 -3.9964 -4.0461 -4.0951 -4.1498 -4.2072 -4.2646 -4.322 -4.3794 -4.4368 -4.4942 -4.5515 -4.61 -4.6685 -4.7269 -4.7854 -4.844 -4.9032 -4.9624 -5.0216 -5.0808 -5.1413 -5.2041 -5.2668 -5.3295 -5.3922 -5.455 -5.5177 -5.5804] % Datasheet derived  OCVChangeThermal=[0, 0; 0, 0; 0, 0; 0, 0] % Parameter not set  R0ChangeVec=[0 0 0 0 0 0 0 0 0 0 0 0 0 0 0 0 0 0 0 0 0 0 0 0 0 0 0 0 0 0 0 0 0 0 0 0 0 0 0 0 0 0 0 0 0 0 0 0 0 0 0 0 0 0 0 0 0 0 0 0 0 0 0 0 0 0 0 0 0 0 0 0 0 0 0 0 0 0 0 0 0 0 0 0] % Parameter assumed  R0ChangeThermal=[0, 0; 0, 0; 0, 0; 0, 0] % Parameter not set  R0ChangeThermalI=repmat(0, 4, 2, 3) % Parameter not set  R0CyclingChangeInitialTarget=0 % Parameter not set  CapacityChangeVec=[0 -0.367 -0.733 -1.1 -1.466 -1.834 -2.202 -2.571 -2.94 -3.309 -3.678 -4.047 -4.261 -4.473 -4.685 -4.897 -5.109 -5.32 -5.532 -5.744 -5.972 -6.21 -6.448 -6.686 -6.924 -7.162 -7.4 -7.638 -7.876 -8.114 -8.313 -8.496 -8.679 -8.862 -9.045 -9.228 -9.411 -9.593 -9.776 -9.959 -10.142 -10.405 -10.679 -10.954 -11.228 -11.503 -11.777 -12.052 -12.326 -12.571 -12.756 -12.941 -13.126 -13.311 -13.496 -13.681 -13.866 -14.051 -14.235 -14.442 -14.659 -14.875 -15.092 -15.308 -15.525 -15.741 -15.958 -16.175 -16.391 -16.607 -16.822 -17.038 -17.254 -17.47 -17.685 -17.901 -18.122 -18.35 -18.579 -18.807 -19.036 -19.265 -19.493 -19.722] % Datasheet derived  CapacityChangeThermal=[0, 0; 0, 0; 0, 0; 0, 0] % Parameter not set  CapacityChangeThermalI=repmat(0, 4, 2, 3) % Parameter not set  CapacityCyclingChangeInitialTarget=0 % Parameter not set  SelfDischargeRChangeVec=[0, 0, 0, 0] % Parameter not set  SelfDischargeRChangeThermal=[0, 0; 0, 0; 0, 0; 0, 0] % Parameter not set  SelfDischargeRChangeThermalI=repmat(0, 4, 2, 3) % Parameter not set  SelfDischargeRCyclingChangeInitialTarget=0 % Parameter not set  R1ChangeVec=[0, 0, 0, 0] % Parameter not set  R1ChangeThermal=[0, 0; 0, 0; 0, 0; 0, 0] % Parameter not set  R1ChangeThermalI=repmat(0, 4, 2, 3) % Parameter not set  R1CyclingChangeInitialTarget=0 % Parameter not set  R2ChangeVec=[0, 0, 0, 0] % Parameter not set  R2ChangeThermal=[0, 0; 0, 0; 0, 0; 0, 0] % Parameter not set  R2ChangeThermalI=repmat(0, 4, 2, 3) % Parameter not set  R2CyclingChangeInitialTarget=0 % Parameter not set  R3ChangeVec=[0, 0, 0, 0] % Parameter not set  R3ChangeThermal=[0, 0; 0, 0; 0, 0; 0, 0] % Parameter not set  R3ChangeThermalI=repmat(0, 4, 2, 3) % Parameter not set  R3CyclingChangeInitialTarget=0 % Parameter not set  CalendarAgeResistance=simscape.battery.enum.cells.BatteryEnable.Disabled  CalendarAgeCapacity=simscape.battery.enum.cells.BatteryEnable.Disabled  CalendarAgingMethod=simscape.battery.enum.cells.CalendarAgingMethod.equation  StorageVariable=simscape.battery.enum.cells.StorageVariable.OCV  OCVDuringStorage=0.9 % Parameter not set  SOCDuringStorage=0.6 % Parameter not set  StorageTimeIntervals=[0] % Parameter not set d  StorageTemperatures=[273] % Parameter not set K  ResistanceScalingOCV=2.2134e6 % Parameter not set  ResistanceScalingOCVOffset=1.632e6 % Parameter not set  ResistanceExponentialIncrease=0.515833569 % Parameter not set V  ResistanceTimeExponent=0.75 % Parameter not set  ResistanceAgeTemperatureBreakpoints=[273.15, 298.15, 323.15] % Parameter not set K  ResistanceAgeTimeBreakpoints=[0, 90, 180, 270] % Parameter not set d  PercentResistanceChange=[0, 0, 0] % Parameter not set  ResistanceTimeBreakpoints=100 % Parameter not set d  PercentResistanceChangeThermal=[0, 0, 0; 0, 0, 0; 0, 0, 0; 0, 0, 0] % Parameter not set  CapacityScalingOCV=1.5097e07 % Parameter not set  CapacityScalingOCVOffset=8.3625e06 % Parameter not set  CapacityExponentialIncrease=0.6011 % Parameter not set V  CapacityTimeExponent=0.75 % Parameter not set  CapacityAgeTemperatureBreakpoints=[273.15, 298.15, 323.15] % Parameter not set K  CapacityAgeTimeBreakpoints=[0, 90, 180, 270] % Parameter not set d  PercentCapacityChange=[0, 0, 0] % Parameter not set  CapacityTimeBreakpoints=100 % Parameter not set d  PercentCapacityChangeThermal=[0, 0, 0; 0, 0, 0; 0, 0, 0; 0, 0, 0] % Parameter not set  SimulationTemperature=298.15 % Parameter not set K  BatteryThermalMass=20.7 % Parameter assumed J/K  NumThermalModels=6 % Parameter not set  ThermalConductivityZ=18 % Parameter not set W/(K*m)  CrossSectionalAreaXY=0.000286 m^2  Height=0.036 m  ReversibleHeatModel=simscape.battery.enum.cells.ReversibleHeatModel.Disabled  EntropicCoefficient=[0, 0, 0, 0, 0, 0, 0] % Parameter not set mV/K  CurrentDirectionality=simscape.battery.enum.cells.BatteryEnable.Disabled  stateOfCharge_specify=off  stateOfCharge_priority=High  stateOfCharge=1  stateOfCharge_nominal_specify=off  stateOfCharge_nominal_value=1  stateOfCharge_nominal_unit=1  batteryVoltage_specify=off  batteryVoltage_priority=Low  batteryVoltage=3 V  batteryVoltage_nominal_specify=off  batteryVoltage_nominal_value=1  batteryVoltage_nominal_unit=V  batteryCurrent_specify=off  batteryCurrent_priority=None  batteryCurrent=0 A  batteryCurrent_nominal_specify=off  batteryCurrent_nominal_value=1  batteryCurrent_nominal_unit=A  numCycles_specify=off  numCycles_priority=High  numCycles=0  numCycles_nominal_specify=off  numCycles_nominal_value=1  numCycles_nominal_unit=1  batteryTemperature_specify=off  batteryTemperature_priority=High  batteryTemperature=298.15 K  batteryTemperature_nominal_specify=off  batteryTemperature_nominal_value=1  batteryTemperature_nominal_unit=K  hysteresisState_specify=off  hysteresisState_priority=High  hysteresisState=0  hysteresisState_nominal_specify=off  hysteresisState_nominal_value=1  hysteresisState_nominal_unit=1  isExothermFaulted_specify=off  isExothermFaulted_priority=None  isExothermFaulted=0  isExothermFaulted_nominal_specify=off  isExothermFaulted_nominal_value=1  isExothermFaulted_nominal_unit=1  reactionHeatRate_specify=off  reactionHeatRate_priority=None  reactionHeatRate=0 W  reactionHeatRate_nominal_specify=off  reactionHeatRate_nominal_value=1  reactionHeatRate_nominal_unit=W  reactionExtent_specify=off  reactionExtent_priority=None  reactionExtent=0  reactionExtent_nominal_specify=off  reactionExtent_nominal_value=1  reactionExtent_nominal_unit=1
      settings: AttributesFormatString=Panasonic:NCA843436  InternalSimscapePortConfiguration="{\"Bottom\":[{\"id\":\"n\",\"label\":\"-\",\"type\":\"foundation.electrical.electrical\"},{\"id\":\"H\",\"label\":\"H\",\"type\":\"foundation.thermal.thermal\"}],\"Left\":[],\"Right\":[],\"Top\":[{\"id\":\"p\",\"label\":\"+\",\"type\":\"foundation.electrical.electrical\"}]}"
  Bias : Bias  Bias=-273.15  SaturateOnIntegerOverflow=off
  Bloco de teste UN38.3 : Subsystem
      settings: PortSchema="{\"entries\":[{\"content\":{\"sides\":[{\"content\":{\"connectorIds\":[\"LConn1\",\"LConn2\"]},\"type\":\"ConnectorPlacement.EquallySpacedRectSide\",\"uuid\":\"b34c29a8-a6a6-4d1f-be7d-5c94c1c9585e\"},{\"content\":{\"connectorIds\":[\"RConn1\",\"RConn2\"],\"side\":\"RIGHT\"},\"type\":\"ConnectorPlacement.EquallySpacedRectSide\",\"uuid\":\"a6deb763-8fbb-4f41-97b4-61744271df4f\"},{\"content\":{\"side\":\"TOP\"},\"type\":\"ConnectorPlacement.EquallySpacedRectSide\",\"uuid\":\"d8cd91aa-967e-429a-9cf9-9069fbc8cbde\"},{\"content\":{\"connectorIds\":[\"RConn3\"],\"side\":\"BOTTOM\"},\"type\":\"ConnectorPlacement.EquallySpacedRectSide\",\"uuid\":\"27e410e3-e66d-40ea-80e4-c4532462ca77\"}]},\"type\":\"ConnectorPlacement.EquallySpacedConnector\",\"uuid\":\"875062d3-ff56-4a82-8ee3-57cc41ca73be\"}],\"packageUris\":[\"http://schema.mathworks.com/mf0/Connector/R2020b\"],\"version\":\"1.0\"}"
  "Coulomb counting " : Subsystem
      settings: PortSchema="{\"entries\":[{\"content\":{\"sides\":[{\"content\":{\"connectorIds\":[\"LConn1\"]},\"type\":\"ConnectorPlacement.EquallySpacedRectSide\",\"uuid\":\"c7cad256-baa2-4d14-bf6b-fa2d40991fde\"},{\"content\":{\"connectorIds\":[\"Out1\",\"RConn1\"],\"side\":\"RIGHT\"},\"type\":\"ConnectorPlacement.EquallySpacedRectSide\",\"uuid\":\"1ac74872-e8be-4cdc-952f-43b6ce73e9dd\"},{\"content\":{\"side\":\"TOP\"},\"type\":\"ConnectorPlacement.EquallySpacedRectSide\",\"uuid\":\"404a2dce-a776-476b-a473-13b33a9ea810\"},{\"content\":{\"connectorIds\":[\"RConn2\"],\"side\":\"BOTTOM\"},\"type\":\"ConnectorPlacement.EquallySpacedRectSide\",\"uuid\":\"6effbad6-327d-4248-b5db-a79e72a2ce8a\"}]},\"type\":\"ConnectorPlacement.EquallySpacedConnector\",\"uuid\":\"fabe5305-7e6e-425a-a397-4bad5b2bd58c\"}],\"packageUris\":[\"http://schema.mathworks.com/mf0/Connector/R2020b\"],\"version\":\"1.0\"}"
  Current Sensor : fl_lib/Electrical/Electrical Sensors/Current Sensor
  Diode{,1..3} (4 alike) : fl_lib/Electrical/Electrical Elements/Diode  Vf=V_direta V  Ron=0.3 Ohm  Goff=1e-8 1/Ohm  i_specify=off  i_priority=None  i=0 A  i_nominal_specify=off  i_nominal_value=1  i_nominal_unit=A  v_specify=off  v_priority=None  v=0 V  v_nominal_specify=off  v_nominal_value=1  v_nominal_unit=V
  Electrical Reference : fl_lib/Electrical/Electrical Elements/Electrical Reference
  Gain : Gain  Gain=1000000
  Ideal Semiconductor Switch : ee_lib/Semiconductors & Converters/Ideal Semiconductor Switch  port_option=ee.enum.controlport.ps  Ron=Rds_on Ohm  Goff=1e-6 1/Ohm  Vth=2.5 V  diode_param=ee.enum.semiconductors.protectionDiode.external  diode_Vf=0.8 V  diode_Ron=0.001 Ohm  diode_Goff=1e-5 1/Ohm  diode_C=50e-9 F  diode_iRM=-235 A  diode_iF=300 A  diode_idot=-50 A/us  diode_trr_param=ee.enum.converters.diodetrr.trr_factor  diode_trr_factor=3  diode_trr=15 us  diode_Qrr=1500 s*uA
  LDO : Subsystem
      settings: PortSchema="{\"entries\":[{\"content\":{\"sides\":[{\"content\":{},\"type\":\"ConnectorPlacement.EquallySpacedRectSide\",\"uuid\":\"f3c1ff26-f66a-474b-908e-c0843d3331d4\"},{\"content\":{\"side\":\"RIGHT\"},\"type\":\"ConnectorPlacement.EquallySpacedRectSide\",\"uuid\":\"ef44fb7d-fd1b-423a-8e0b-edc78d3f1410\"},{\"content\":{\"connectorIds\":[\"LConn1\"],\"side\":\"TOP\"},\"type\":\"ConnectorPlacement.EquallySpacedRectSide\",\"uuid\":\"e3d6ea15-9f85-4f8b-8e1d-58ef3823ceb2\"},{\"content\":{\"connectorIds\":[\"RConn1\"],\"side\":\"BOTTOM\"},\"type\":\"ConnectorPlacement.EquallySpacedRectSide\",\"uuid\":\"e25aef70-2430-4641-87c0-edb84bfaa03b\"}]},\"type\":\"ConnectorPlacement.EquallySpacedConnector\",\"uuid\":\"d37bc179-a1f5-4208-842c-e06ccf67eb47\"}],\"packageUris\":[\"http://schema.mathworks.com/mf0/Connector/R2020b\"],\"version\":\"1.0\"}"
  Mux : Mux  Inputs=2
  PPTC FUSE : Subsystem
  PPTC FUSE1 : Subsystem
  PPTC FUSE2 : Subsystem
  PPTC FUSE3 : Subsystem
  PS-Simulink Converter{,1..3} (4 alike) : nesl_utility/PS-Simulink Converter  PhysicalDomain=network_engine_domain  SubClassName=ps_output  LeftPortType=input  RightPortType=output  PseudoPeriodic=off  Frequencies=[]  VectorFormat=inherit  Unit=inherit  AffineConversion=off
  Saída do teste : Scope  NumInputPorts=2
      settings: ActiveDisplayYMinimum=24.999622633700163  ActiveDisplayYMaximum=25.003396296698533  DataLoggingVariableName=ScopeData2
  Scope : Scope
      settings: ActiveDisplayYMinimum=0.59237854983928862  ActiveDisplayYMaximum=1.0048888623395469
  Scope1 : Scope
      settings: ActiveDisplayYMinimum=3  ActiveDisplayYMaximum=203  DataLoggingVariableName=ScopeData3
  Solver Configuration : nesl_utility/Solver Configuration  PhysicalDomain=network_engine_domain  SubClassName=solver  LeftPortType=input  RightPortType=generic  Tones=[]  Harmonics=[]  SimulateNoise=off  Profile=off  UseLocalSampling=off  EnableSwitchedLinearOptims=on  FrequencyDomain=off  UseCCode=off  RelTol=0.001  AbsTol=0.001  MinStep=1e-09  ToWorkspace=off  RevertToSquareIcSolve=off  NumHomotopyIterations=100  PhasorMode=off  PhasorModeNumHarmonics=1  ConsistencySolver=NEWTON_XTOL_AFTER_FTOL  IndexReductionMethod=DerivativeReplacement  DoDC=off  ResidualTolerance=1e-09  ConsistencyTolSource=GLOBAL  ConsistencyAbsTol=0.001  ConsistencyRelTol=0.001  ConsistencyTolFactor=0.001  UseLocalSolver=off  LocalSolverChoice=NE_BACKWARD_EULER_ADVANCER  ResolveIndetEquations=on  FunctionEvalNumThread=1  LocalSolverSampleTime=0.001  DoFixedCost=off  MaxNonlinIter=3  MaxModeIter=2  ComputeImpulses=off  ImpulseIterations=2  LinearAlgebra=auto  LinearAlgebraNumThread=0  EquationFormulation=NE_TIME_EF  DelaysMemoryBudget=1024  AutomaticFiltering=on  FilteringTimeConstant=0.01  PartitionStorageMethod=AS_NEEDED  PartitionMemoryBudget=1024  PartitionMethod=ROBUST  MultibodyUseLocalSolver=off  MultibodyLocalSolverChoice=ODE1  MultibodyLocalSolverSampleTime=0.001
  Temperature Sensor : fl_lib/Thermal/Thermal Sensors/Temperature Sensor  temperature_measure=foundation.enum.MeasurementReference.difference
  Thermal Reference : fl_lib/Thermal/Thermal Elements/Thermal Reference
  Thermal Switch : Subsystem
      settings: PortSchema="{\"entries\":[{\"content\":{\"sides\":[{\"content\":{},\"type\":\"ConnectorPlacement.EquallySpacedRectSide\",\"uuid\":\"26343e8b-9037-463a-8d52-b8aa2b4784ac\"},{\"content\":{\"side\":\"RIGHT\"},\"type\":\"ConnectorPlacement.EquallySpacedRectSide\",\"uuid\":\"97dbbb4c-3f50-4fbe-907b-6f17cf04a957\"},{\"content\":{\"connectorIds\":[\"LConn1\",\"LConn2\"],\"side\":\"TOP\"},\"type\":\"ConnectorPlacement.EquallySpacedRectSide\",\"uuid\":\"784a0f5a-ad9e-41a1-b3aa-064eb583841a\"},{\"content\":{\"connectorIds\":[\"In1\",\"RConn1\"],\"side\":\"BOTTOM\"},\"type\":\"ConnectorPlacement.EquallySpacedRectSide\",\"uuid\":\"beca7415-8e69-424c-bf78-cdc77b2f5ca2\"}]},\"type\":\"ConnectorPlacement.EquallySpacedConnector\",\"uuid\":\"dd282009-0dac-47f7-a447-bdd8e97d6e76\"}],\"packageUris\":[\"http://schema.mathworks.com/mf0/Connector/R2020b\"],\"version\":\"1.0\"}"
  wires:
  Bias/1 -> Saída do teste/2, Thermal Switch/1(Temp)
  PS-Simulink Converter2/1 -> Bias/1
  "Coulomb counting "/1(SOC) -> Scope/1
  PS-Simulink Converter1/1 -> Mux/2
  PS-Simulink Converter/1 -> Mux/1
  Mux/1 -> Saída do teste/1
  PS-Simulink Converter3/1 -> Gain/1
  Gain/1 -> Scope1/1
  connections:
  Battery Equivalent Circuit/LConn1 -- Diode/LConn1
  "Coulomb counting "/RConn2 -- Bloco de teste UN38.3/LConn2 -- Thermal Switch/RConn1 -- LDO/RConn1 -- Battery Equivalent Circuit8/RConn1 -- Battery Equivalent Circuit9/RConn1 -- Battery Equivalent Circuit10/RConn1 -- Battery Equivalent Circuit11/RConn1 -- Solver Configuration/RConn1 -- Electrical Reference/LConn1
  Temperature Sensor/RConn2 -- PS-Simulink Converter2/LConn1
  Thermal Reference/LConn1 -- Temperature Sensor/RConn1
  PPTC FUSE1/RConn1 -- PPTC FUSE3/RConn1 -- PPTC FUSE2/RConn1 -- Current Sensor/LConn1 -- PPTC FUSE/RConn1
  PPTC FUSE/LConn1 -- Diode/RConn1
  Temperature Sensor/LConn1 -- Bloco de teste UN38.3/RConn3 -- Battery Equivalent Circuit11/RConn2 -- Battery Equivalent Circuit7/RConn2 -- Battery Equivalent Circuit3/RConn2 -- Battery Equivalent Circuit10/RConn2 -- Battery Equivalent Circuit6/RConn2 -- Battery Equivalent Circuit9/RConn2 -- Battery Equivalent Circuit5/RConn2 -- Battery Equivalent Circuit8/RConn2 -- Battery Equivalent Circuit4/RConn2 -- Battery Equivalent Circuit/RConn2 -- Battery Equivalent Circuit1/RConn2 -- Battery Equivalent Circuit2/RConn2
  Diode3/LConn1 -- Battery Equivalent Circuit3/LConn1
  Diode2/LConn1 -- Battery Equivalent Circuit2/LConn1
  Diode1/LConn1 -- Battery Equivalent Circuit1/LConn1
  Diode1/RConn1 -- PPTC FUSE1/LConn1
  Diode2/RConn1 -- PPTC FUSE2/LConn1
  Diode3/RConn1 -- PPTC FUSE3/LConn1
  Thermal Switch/LConn1 -- LDO/LConn1 -- "Coulomb counting "/RConn1 -- Ideal Semiconductor Switch/RConn1
  Battery Equivalent Circuit3/RConn1 -- Battery Equivalent Circuit7/LConn1
  Battery Equivalent Circuit2/RConn1 -- Battery Equivalent Circuit6/LConn1
  Battery Equivalent Circuit1/RConn1 -- Battery Equivalent Circuit5/LConn1
  Battery Equivalent Circuit/RConn1 -- Battery Equivalent Circuit4/LConn1
  Battery Equivalent Circuit8/LConn1 -- Battery Equivalent Circuit4/RConn1
  Battery Equivalent Circuit9/LConn1 -- Battery Equivalent Circuit5/RConn1
  Battery Equivalent Circuit10/LConn1 -- Battery Equivalent Circuit6/RConn1
  Battery Equivalent Circuit11/LConn1 -- Battery Equivalent Circuit7/RConn1
  Thermal Switch/LConn2 -- Ideal Semiconductor Switch/LConn1
  Bloco de teste UN38.3/LConn1 -- Ideal Semiconductor Switch/RConn2
  PS-Simulink Converter/LConn1 -- Bloco de teste UN38.3/RConn1
  PS-Simulink Converter1/LConn1 -- Bloco de teste UN38.3/RConn2
  Current Sensor/RConn2 -- "Coulomb counting "/LConn1
  Current Sensor/RConn1 -- PS-Simulink Converter3/LConn1
